simulink model "modelo_BDA"  (R2021b)
settings: Solver=ode3  StartTime=0.0  StopTime=10.0  FixedStep=1e-6  RelTol=1e-3
(part 2 of 4)

== matlab function modelo_BDA/h ==
  data: dq input; h output double; q input
function h = h(dq,q)
%#codegen
dq1 = dq(1);
dq2 = dq(2);
dq3 = dq(3);
dq4 = dq(4);
dq5 = dq(5);
dq6 = dq(6);

q1 = q(1);
q2 = q(2);
q3 = q(3);
q4 = q(4);
q5 = q(5);
q6 = q(6);
%    This function was generated by the Symbolic Math Toolbox version 9.0.
%    01-Dec-2021 19:55:05

t2 = cos(q1);
t3 = cos(q2);
t4 = cos(q4);
t5 = cos(q5);
t6 = cos(q6);
t7 = sin(q1);
t8 = sin(q2);
t9 = sin(q4);
t10 = sin(q5);
t11 = sin(q6);
t12 = dq1+dq2;
t13 = dq5.*6.0;
t20 = dq6.*7.26735103;
t21 = dq1.*2.038587093e+1;
t22 = dq2.*2.038587093e+1;
t23 = dq4.*2.889644336e+1;
t28 = dq5.*1.087689656e+1;
t29 = dq3.*5.110348748545983e-1;
t33 = dq3.*8.595599785252598e-1;
t34 = 9.007199254740992e+15;
t48 = dq6.*1.336375981993753e+2;
t50 = dq6.*7.263507131821755e+1;
t52 = dq4.*6.678442840618982e+2;
t53 = dq5.*6.185536839278779e+1;
t54 = dq5.*1.356524863046341e+2;
t56 = dq4.*1.688943762888624e+2;
t59 = dq3.*1.476709031622059e+1;
t61 = dq3.*1.705746846438843;
t62 = dq5.*7.051076542399408e-1;
t63 = dq3.*2.869063922714997;
t65 = dq4.*1.870703729528352e-1;
t66 = dq6.*1.40259874879e-5;
t84 = dq6.*1.246862890394724e+3;
t87 = dq4.*6.597219446016286e+2;
t88 = dq5.*7.291450524218959e+2;
t90 = dq3.*3.41291720127931e+2;
t94 = dq3.*8.631091645042425e+1;
t99 = dq4.*2.625724653752266e+4;
t100 = dq5.*2.524704765397172;
t101 = dq3.*1.573543358425071e+1;
t103 = dq5.*1.758766552463174e+1;
t104 = dq4.*4.967071763045598;
t105 = dq3.*2.942260910305135e+1;
t109 = dq3.*4.515804268730207e+1;
t110 = dq3.*9.559948463095517e-2;
t111 = dq3.*2.64669783204376e+1;
t112 = dq3.*1.74926470944712e+1;
t116 = dq6.*4.126305645247942e-4;
t117 = dq6.*3.146556876441599e-4;
t118 = dq4.*1.692526621106363;
t124 = dq3.*1.483306048043653e-5;
t125 = dq3.*8.818711196088817e-6;
t126 = dq5.*5.878411097842592e+2;
t127 = dq5.*2.257319383180457e+3;
t129 = dq4.*2.326738990698287e+4;
t130 = dq6.*1.744166601788531e+3;
t131 = dq6.*3.383303336574349e+3;
t132 = dq3.*3.371409213983255e+2;
t135 = dq3.*4.384438618576911e+2;
t138 = dq3.*7.374619913957088e+2;
t147 = dq3.*2.538346896821816;
t148 = dq3.*1.341836869832923e+4;
t150 = dq3.*8.649401300051666e-1;
t162 = dq3.*5.644976860104108e-5;
t163 = dq3.*4.471679626929696e-4;
t164 = dq3.*2.65855123043135e-4;
t165 = dq3.*9.494843556473991e-5;
t166 = dq3.*3.907181940919286e-4;
t171 = dq3.*1.189044768930814e+4;
t176 = dq3.*4.580783722140037e+2;
t177 = dq3.*5.353365437196861e+2;
t14 = t12.^2;
t15 = t2.*t3.*9.81e+3;
t16 = t2.*t8.*9.81e+3;
t17 = t3.*t7.*9.81e+3;
t18 = t7.*t8.*9.81e+3;
t24 = t3.*3.235524933e+1;
t25 = t8.*3.235524933e+1;
t26 = t3.*1.0513390433e+2;
t27 = t8.*1.0513390433e+2;
t30 = t5.*5.110348748545983e-1;
t32 = t10.*5.110348748545983e-1;
t35 = t5.*t9.*8.595599785252598e-1;
t36 = t9.*t10.*8.595599785252598e-1;
t38 = (q3.*t34)./9.007199254740992e+15;
t41 = q3.*t34.*1.110223024625157e-16i;
t67 = -t62;
t68 = t21+t22;
t69 = t7.*t8.*4.486343276457132e+6;
t70 = t2.*t8.*3.161091753815448e+6;
t71 = t3.*t7.*3.161091753815448e+6;
t73 = t2.*t3.*4.486343276457132e+6;
t113 = -t103;
t115 = -t105;
t128 = -t126;
t168 = -t163;
t19 = -t18;
t31 = -t27;
t37 = -t36;
t39 = cos(t38);
t40 = sin(t38);
t42 = exp(t41);
t44 = -t41;
t72 = t25+t26;
t74 = -t69;
t75 = -t70;
t76 = -t71;
t80 = t32+t35;
t43 = t39.^2;
t45 = 1.0./t42;
t46 = t4.*t39;
t47 = t9.*t39;
t51 = t42-1.0;
t77 = t24+t31;
t78 = dq1.*dq2.*t72;
t81 = t30+t37;
t83 = t39.*1.318958611e+1;
t120 = t5.*t12.*t33.*t39;
t122 = t10.*t12.*t33.*t39;
t123 = dq3.*t5.*t12.*t39.*(-8.595599785252598e-1);
t137 = t42.*3.694216783411725e-1;
t145 = t42.*1.305783216588275e-1;
t161 = t12.*t39.*1.72565741205e-5;
t172 = t4.*t34.*t40.*5.673626844500105e-17;
t173 = t9.*t34.*t40.*5.673626844500105e-17;
t174 = t5.*t34.*t40.*9.543032792050485e-17;
t175 = t10.*t34.*t40.*9.543032792050485e-17;
t178 = t4.*t34.*t40.*3.404176106700063e-16;
t181 = t12.*t34.*t40.*5.673626844500105e-17;
t182 = t12.*t34.*t40.*9.543032792050485e-17;
t184 = t42.*3.269483204543573;
t189 = t42.*1.334999662191606e+1;
t192 = t12.*t39.*2.666747250761074e+2;
t193 = dq3.*t10.*t12.*t39.*6.243420034246779e+1;
t196 = dq3.*t12.*t39.*1.451748464558917e+2;
t198 = dq3.*t10.*t12.*t39.*1.148695310384223e+2;
t200 = t12.*t39.*t109;
t202 = dq3.*t10.*t12.*t39.*5.316839912737671e+1;
t212 = dq3.*t12.*t39.*(-4.515804268730207e+1);
t216 = dq3.*t5.*t12.*t39.*1.166014482149094e+2;
t222 = dq3.*t12.*t39.*1.607982057580514e-1;
t227 = t12.*t39.*1.104616756676389e-4;
t228 = dq3.*t5.*t12.*t39.*6.060823201364798e-1;
t229 = dq3.*t10.*t12.*t39.*6.060823201364798e-1;
t230 = t12.*t39.*5.202289239433555e-4;
t231 = t12.*t39.*t125;
t232 = t12.*t39.*t124;
t241 = t4.*t34.*t40.*2.556183965391409e-15;
t242 = t34.*t40.*4.869208971920574e-15;
t243 = t9.*t34.*t40.*9.827649182848514e-15;
t244 = t9.*t34.*t40.*4.958440210927941e-15;
t246 = t4.*t34.*t40.*7.425392937311983e-15;
t248 = t12.*t39.*4.478274624984646e+2;
t249 = t12.*t39.*4.642566765942165e+2;
t250 = t12.*t34.*t40.*2.757597065581095e-15;
t251 = t12.*t34.*t40.*3.18530082611956e-16;
t252 = t12.*t34.*t40.*1.893759423098155e-16;
t256 = dq3.*t12.*t39.*5.670705805344185e+2;
t263 = dq3.*t5.*t12.*t39.*6.267439056015643e+2;
t264 = dq3.*t10.*t12.*t39.*3.610943527871318e+3;
t265 = dq3.*t10.*t12.*t39.*6.267439056015643e+2;
t273 = dq3.*t12.*t39.*4.269496097976898;
t278 = dq3.*t5.*t12.*t39.*2.170135173927414;
t287 = dq3.*t10.*t12.*t39.*1.511765340066191e+1;
t288 = t12.*t39.*t166;
t289 = dq3.*t10.*t12.*t39.*3.54680719181798e-4;
t290 = dq3.*t10.*t12.*t39.*2.704654361142649e-4;
t292 = dq3.*t5.*t12.*t39.*1.940301400531246e+3;
t293 = dq3.*t10.*t12.*t39.*5.052846917024227e+2;
t294 = dq3.*t12.*t39.*3.522681996322863e+3;
t296 = t12.*t34.*t40.*6.373259902786174e-14;
t297 = t12.*t34.*t40.*1.611764571317528e-14;
t298 = t12.*t34.*t40.*1.74698406676951e-15;
t299 = t12.*t34.*t40.*1.942073956592427e-15;
t301 = t12.*t34.*t40.*1.78521870351002e-17;
t303 = t12.*t39.*t176;
t304 = t12.*t34.*t40.*3.266565807075334e-15;
t305 = t12.*t39.*t177;
t306 = t12.*t34.*t40.*2.938424872360468e-15;
t307 = t12.*t34.*t40.*9.963509157680404e-16;
t309 = dq3.*t12.*t39.*(-5.353365437196861e+2);
t312 = t12.*t34.*t40.*9.790736217417458e-22;
t315 = t12.*t34.*t40.*1.646800527103812e-21;
t318 = t34.*t40.*t72.*5.673626844500105e-17;
t344 = t12.*t34.*t40.*4.867704704399801e-14;
t345 = t12.*t34.*t40.*8.18747282633435e-14;
t346 = t12.*t34.*t40.*6.295748150968656e-14;
t348 = t12.*t34.*t40.*2.505737647365328e-12;
t350 = t12.*t34.*t40.*4.740092871521216e-16;
t351 = t12.*t34.*t40.*6.267183283563802e-21;
t352 = t12.*t34.*t40.*1.054139393161123e-20;
t353 = t12.*t34.*t40.*1.615183704663643e-16;
t355 = t12.*t34.*t40.*2.951584788170425e-20;
t357 = t12.*t34.*t40.*4.005724181331548e-20;
t358 = t12.*t34.*t40.*4.964561680564579e-20;
t375 = t12.*t34.*t40.*2.220414648677621e-12;
t402 = t12.*t34.*t40.*8.913349685100906e-16;
t406 = t12.*t34.*t40.*2.760619280862119e-14;
t49 = t47.*6.0;
t55 = t12.*t46;
t57 = t12.*t47;
t58 = t51.^2;
t79 = dq1.*dq2.*t77;
t85 = t46.*2.286892447e+1;
t86 = t47.*2.286892447e+1;
t89 = t12.*t83;
t91 = t46.*6.520967601e+1;
t92 = t15+t19+t78;
t146 = t45.*3.694216783411725e-1;
t152 = t45.*1.305783216588275e-1;
t155 = t14.*t43.*3.422984996757468e+1;
t157 = t14.*t43.*3.079131064925427e+1;
t167 = -t161;
t169 = t78.*4.573234736449676e+2;
t179 = -t173;
t180 = -t174;
t183 = -t181;
t185 = t45.*3.269483204543573;
t195 = t45.*1.334999662191606e+1;
t199 = -t192;
t201 = -t193;
t204 = -t196;
t223 = -t216;
t245 = -t243;
t247 = t12.*t242;
t253 = -t252;
t254 = t29+t182;
t267 = -t263;
t268 = -t264;
t269 = -t265;
t277 = -t273;
t291 = -t290;
t300 = -t298;
t302 = t47+t172;
t316 = -t312;
t319 = t34.*t40.*t77.*9.543032792050485e-17;
t320 = dq1.*t318;
t325 = dq1.*t34.*t40.*t77.*(-9.543032792050485e-17);
t347 = -t344;
t356 = -t351;
t361 = -t357;
t363 = t61+t251;
t403 = -t402;
t417 = t23+t59+t250;
t491 = t112+t304;
t492 = t109+t307;
t502 = t125+t315;
t604 = t56+t94+t297;
t610 = t65+t110+t301;
t624 = t176+t406;
t630 = t115+t161+t299;
t701 = t135+t230+t345;
t704 = t168+t192+t355;
t746 = t164+t249+t358;
t60 = t12.*t49;
t64 = -t57;
t82 = -t79;
t93 = -t91;
t95 = t55.*2.889644336e+1;
t96 = t57.*2.889644336e+1;
t97 = t55.*2.286892447e+1;
t98 = t57.*2.286892447e+1;
t102 = t55.*6.520967601e+1;
t107 = t57.*1.087689656e+1;
t114 = t29.*t57;
t119 = t29.*t55;
t121 = dq3.*t57.*(-5.110348748545983e-1);
t133 = t55.*6.678442840618982e+2;
t134 = t57.*6.678442840618982e+2;
t136 = dq3.*t55.*2.302405830805438e+1;
t139 = t57.*6.185536839278779e+1;
t140 = t55.*1.688943762888624e+2;
t141 = dq3.*t55.*2.228321894484292e+1;
t142 = t57.*1.356524863046341e+2;
t143 = t57.*1.688943762888624e+2;
t149 = dq3.*t57.*4.466165897254792e+1;
t153 = t57.*7.051076542399408e-1;
t154 = t55.*1.870703729528352e-1;
t156 = t57.*1.870703729528352e-1;
t170 = t79.*3.22231575312482e+2;
t186 = t55.*6.597219446016286e+2;
t187 = t57.*6.597219446016286e+2;
t188 = t57.*7.291450524218959e+2;
t191 = dq3.*t55.*4.097608396301209e+2;
t194 = dq3.*t55.*2.227143274869608e+2;
t197 = dq3.*t57.*4.857802448423996e+2;
t203 = t57.*t94;
t206 = t57.*2.625724653752266e+4;
t207 = dq3.*t55.*3.161025044569338e+1;
t208 = dq3.*t55.*6.932315136240378e+1;
t209 = t57.*2.524704765397172;
t210 = dq3.*t55.*1.006605116943962e+3;
t211 = dq3.*t57.*1.006605116943962e+3;
t213 = t57.*1.758766552463174e+1;
t214 = t55.*4.967071763045598;
t215 = t57.*4.967071763045598;
t224 = t55.*1.692526621106363;
t225 = t57.*1.692526621106363;
t226 = t55.*t110;
t233 = t57.*5.878411097842592e+2;
t234 = t57.*2.257319383180457e+3;
t236 = t55.*4.098238731829628e+3;
t237 = t57.*4.098238731829628e+3;
t238 = t55.*2.326738990698287e+4;
t255 = dq4+t254;
t257 = t33+t183;
t258 = dq3.*t55.*1.359241913128349e+3;
t259 = dq3.*t57.*6.058465082115794e+3;
t260 = dq3.*t57.*2.762563368780008e+3;
t270 = dq3.*t55.*4.225774888975571e+3;
t276 = dq3.*t57.*2.87948544352712e+4;
t279 = dq3.*t57.*6.845466071397372;
t280 = dq3.*t55.*8.987910450364716;
t281 = dq3.*t55.*1.290212183829552;
t282 = t55.*t150;
t283 = t57.*t150;
t295 = dq3.*t55.*2.726693342625011e+4;
t308 = t46+t179;
t310 = t6.*t302;
t311 = t11.*t302;
t321 = -t319;
t322 = dq1.*t319;
t323 = t4.*t254.*1.318958611e+1;
t324 = t9.*t254.*1.318958611e+1;
t328 = t33.*t254;
t330 = t45.*t58.*5.499266393288274;
t332 = dq3.*t254.*(-8.595599785252598e-1);
t341 = t45.*t58.*7.936984065608979;
t349 = t34.*t40.*t92.*9.543032792050485e-17;
t360 = t5.*t302.*4.234075154e+1;
t362 = t10.*t302.*4.234075154e+1;
t364 = t63+t253;
t367 = dq3.*t254.*1.133724035346867e+1;
t408 = t45.*t58.*t72.*2.196325630278387e-1;
t409 = t45.*t58.*t77.*2.196325630278387e-1;
t413 = dq1.*t45.*t58.*t77.*(-2.196325630278387e-1);
t414 = t34.*t40.*t92.*3.18530082611956e-16;
t418 = dq3.*t254.*3.276059237327137e+2;
t429 = t105.*t254;
t431 = t111.*t254;
t435 = dq3.*t254.*(-2.64669783204376e+1);
t458 = t45.*t58.*t92.*2.196325630278387e-1;
t482 = t34.*t40.*t92.*3.266565807075334e-15;
t483 = t34.*t40.*t92.*2.938424872360468e-15;
t490 = t111+t300;
t493 = dq3.*t254.*1.914796138336013e+3;
t495 = t138.*t254;
t497 = dq3.*t254.*2.120861781179316;
t503 = t165.*t254;
t504 = t163.*t254;
t505 = t124+t316;
t506 = dq3.*t254.*(-9.494843556473991e-5);
t508 = dq3.*t254.*(-4.471679626929696e-4);
t517 = t45.*t58.*t92.*7.330958613472507e-1;
t531 = t137+t146+2.61156643317655e-1;
t536 = t145+t152+7.38843356682345e-1;
t551 = t45.*t58.*t92.*6.762774476882097;
t577 = t45.*t58.*t92.*3.790105603165286e-6;
t605 = t12.*t39.*t492;
t613 = t166+t361;
t623 = t177+t403;
t628 = t101+t167+t306;
t668 = t254.*t491;
t670 = t254.*t502;
t702 = t138+t227+t347;
t703 = t162+t199+t352;
t745 = t165+t248+t356;
t756 = t12.*t39.*t701;
t765 = t247+t320+t325;
t769 = t254.*t630;
t800 = t254.*t704;
t806 = t254.*t746;
t106 = t16+t17+t82;
t108 = -t96;
t144 = -t134;
t151 = -t143;
t158 = -t153;
t159 = -t154;
t160 = -t156;
t190 = -t187;
t205 = -t197;
t217 = -t210;
t218 = -t211;
t219 = -t213;
t220 = -t214;
t221 = -t215;
t235 = -t233;
t239 = -t236;
t240 = -t237;
t261 = t5.*t255;
t262 = t10.*t255;
t266 = -t260;
t271 = t4.*t257;
t272 = t9.*t257;
t286 = -t279;
t313 = t5.*t308;
t314 = t10.*t308;
t317 = -t311;
t327 = -t324;
t331 = t29.*t257;
t372 = dq3.*t257.*6.740338487107798;
t410 = dq1.*t408;
t411 = -t409;
t412 = dq1.*t409;
t415 = -t414;
t424 = dq3.*t257.*1.947718093199386e+2;
t436 = t101.*t257;
t438 = t112.*t257;
t448 = dq3.*t257.*(-1.74926470944712e+1);
t460 = -t458;
t485 = -t482;
t494 = dq3.*t257.*1.138405264755886e+3;
t498 = t135.*t257;
t499 = dq3.*t257.*(-4.384438618576911e+2);
t500 = dq3.*t257.*1.260917634611605;
t507 = t162.*t257;
t514 = t164.*t257;
t557 = -t551;
t583 = -t577;
t617 = t72.*t536;
t618 = t77.*t531;
t625 = t92.*t531;
t629 = t12.*t39.*t613;
t669 = t257.*t490;
t671 = t257.*t505;
t744 = t255.*t604;
t747 = t255.*t610;
t757 = t12.*t39.*t702;
t758 = -t756;
t759 = t254.*t623;
t761 = t257.*t624;
t762 = t242+t318+t321;
t766 = t4.*t765;
t767 = t9.*t765;
t770 = t184+t185+t341+1.849951749091285e+1;
t771 = t257.*t628;
t775 = t189+t195+t330+9.437562846167879;
t784 = t29.*t765;
t785 = t33.*t765;
t786 = dq3.*t765.*2.483822623397798e+1;
t787 = t63.*t765;
t788 = t61.*t765;
t789 = dq3.*t765.*(-1.705746846438843);
t793 = dq3.*t765.*1.451748464558917e+2;
t794 = t109.*t765;
t796 = dq3.*t765.*1.607982057580514e-1;
t797 = t124.*t765;
t799 = t125.*t765;
t801 = t257.*t703;
t807 = t12.*t39.*t765.*3.422984996757468e+1;
t808 = t12.*t39.*t765.*3.079131064925427e+1;
t809 = t257.*t745;
t837 = t363.*t765;
t838 = t364.*t765;
t893 = t492.*t765;
t274 = -t261;
t275 = t271.*6.0;
t284 = -t271;
t326 = t262.*7.26735103;
t329 = t262.*1.087689656e+1;
t333 = t271.*2.889644336e+1;
t334 = t272.*2.889644336e+1;
t335 = t271.*2.286892447e+1;
t336 = t272.*2.286892447e+1;
t337 = t261.*1.087689656e+1;
t338 = t272.*6.520967601e+1;
t339 = t271.*1.087689656e+1;
t354 = t34.*t40.*t106.*5.673626844500105e-17;
t365 = t262.*7.263507131821755e+1;
t366 = t262.*1.336375981993753e+2;
t368 = t272.*6.678442840618982e+2;
t369 = t261.*1.356524863046341e+2;
t370 = t262.*1.356524863046341e+2;
t371 = t261.*6.185536839278779e+1;
t373 = t262.*6.185536839278779e+1;
t374 = t271.*6.678442840618982e+2;
t377 = t271.*6.185536839278779e+1;
t379 = t271.*1.356524863046341e+2;
t380 = -t372;
t381 = t271.*1.688943762888624e+2;
t382 = t272.*1.688943762888624e+2;
t383 = t261.*7.051076542399408e-1;
t384 = t262.*7.051076542399408e-1;
t389 = t271.*7.051076542399408e-1;
t390 = t262.*1.40259874879e-5;
t391 = t55+t272;
t392 = t271.*1.870703729528352e-1;
t393 = t272.*1.870703729528352e-1;
t396 = t64+t271;
t416 = t34.*t40.*t106.*1.893759423098155e-16;
t419 = t261.*7.291450524218959e+2;
t420 = t262.*7.291450524218959e+2;
t421 = t262.*1.246862890394724e+3;
t422 = t261.*2.65978307941329e+3;
t423 = t262.*2.65978307941329e+3;
t426 = t271.*6.597219446016286e+2;
t427 = t271.*7.291450524218959e+2;
t428 = t272.*6.597219446016286e+2;
t430 = -t424;
t433 = t261.*2.524704765397172;
h = ft_1({dq1,dq2,dq3,dq4,dq5,dq6,t10,t100,t101,t102,t103,t104,t105,t106,t107,t108,t11,t111,t112,t113,t116,t117,t118,t119,t12,t120,t121,t122,t123,t126,t127,t128,t129,t13,t130,t131,t132,t133,t134,t136,t139,t140,t141,t142,t143,t144,t147,t148,t149,t150,t151,t153,t154,t155,t156,t157,t158,t159,t160,t169,t170,t171,t174,t175,t178,t180,t186,t188,t190,t191,t194,t196,t197,t198,t2,t20,t201,t202,t203,t204,t205,t206,t207,t208,t209,t210,t211,t212,t215,t216,t217,t218,t219,t220,t221,t222,t223,t224,t225,t226,t228,t229,t23,t231,t232,t234,t235,t238,t239,t240,t241,t244,t245,t246,t254,t255,t256,t257,t258,t259,t261,t262,t264,t266,t267,t268,t269,t270,t271,t272,t274,t275,t276,t277,t278,t28,t280,t281,t282,t283,t284,t286,t287,t288,t289,t29,t291,t292,t293,t294,t295,t296,t3,t302,t303,t305,t308,t309,t310,t311,t313,t314,t317,t323,t326,t327,t328,t329,t33,t331,t332,t333,t334,t335,t336,t337,t338,t339,t34,t346,t348,t349,t350,t353,t354,t360,t362,t363,t364,t365,t366,t367,t368,t369,t370,t371,t373,t374,t375,t377,t379,t380,t381,t382,t383,t384,t389,t39,t390,t391,t392,t393,t4,t40,t408,t410,t411,t413,t415,t416,t417,t418,t419,t420,t421,t422,t423,t426,t427,t428,t429,t430,t433,t435,t436,t448,t45,t460,t48,t482,t483,t485,t49,t490,t491,t493,t494,t495,t497,t499,t5,t50,t500,t502,t504,t505,t506,t507,t508,t514,t517,t52,t53,t536,t54,t55,t557,t56,t57,t577,t58,t583,t6,t60,t604,t605,t61,t610,t617,t618,t62,t625,t628,t629,t63,t630,t65,t66,t668,t669,t67,t670,t671,t68,t7,t72,t73,t74,t744,t747,t75,t756,t757,t758,t759,t76,t761,t762,t765,t766,t767,t769,t77,t770,t771,t775,t78,t784,t785,t786,t787,t789,t79,t793,t794,t796,t797,t799,t8,t80,t800,t801,t806,t807,t808,t809,t81,t83,t837,t838,t84,t85,t86,t87,t88,t89,t893,t9,t90,t91,t92,t93,t95,t96,t97,t98,t99});
end
function h = ft_1(ct)
dq1 = ct{1};
dq2 = ct{2};
dq3 = ct{3};
dq4 = ct{4};
dq5 = ct{5};
dq6 = ct{6};
t10 = ct{7};
t100 = ct{8};
t101 = ct{9};
t102 = ct{10};
t103 = ct{11};
t104 = ct{12};
t105 = ct{13};
t106 = ct{14};
t107 = ct{15};
t108 = ct{16};
t11 = ct{17};
t111 = ct{18};
t112 = ct{19};
t113 = ct{20};
t116 = ct{21};
t117 = ct{22};
t118 = ct{23};
t119 = ct{24};
t12 = ct{25};
t120 = ct{26};
t121 = ct{27};
t122 = ct{28};
t123 = ct{29};
t126 = ct{30};
t127 = ct{31};
t128 = ct{32};
t129 = ct{33};
t13 = ct{34};
t130 = ct{35};
t131 = ct{36};
t132 = ct{37};
t133 = ct{38};
t134 = ct{39};
t136 = ct{40};
t139 = ct{41};
t140 = ct{42};
t141 = ct{43};
t142 = ct{44};
t143 = ct{45};
t144 = ct{46};
t147 = ct{47};
t148 = ct{48};
t149 = ct{49};
t150 = ct{50};
t151 = ct{51};
t153 = ct{52};
t154 = ct{53};
t155 = ct{54};
t156 = ct{55};
t157 = ct{56};
t158 = ct{57};
t159 = ct{58};
t160 = ct{59};
t169 = ct{60};
t170 = ct{61};
t171 = ct{62};
t174 = ct{63};
t175 = ct{64};
t178 = ct{65};
t180 = ct{66};
t186 = ct{67};
t188 = ct{68};
t190 = ct{69};
t191 = ct{70};
t194 = ct{71};
t196 = ct{72};
t197 = ct{73};
t198 = ct{74};
t2 = ct{75};
t20 = ct{76};
t201 = ct{77};
t202 = ct{78};
t203 = ct{79};
t204 = ct{80};
t205 = ct{81};
t206 = ct{82};
t207 = ct{83};
t208 = ct{84};
t209 = ct{85};
t210 = ct{86};
t211 = ct{87};
t212 = ct{88};
t215 = ct{89};
t216 = ct{90};
t217 = ct{91};
t218 = ct{92};
t219 = ct{93};
t220 = ct{94};
t221 = ct{95};
t222 = ct{96};
t223 = ct{97};
t224 = ct{98};
t225 = ct{99};
t226 = ct{100};
t228 = ct{101};
t229 = ct{102};
t23 = ct{103};
t231 = ct{104};
t232 = ct{105};
t234 = ct{106};
t235 = ct{107};
t238 = ct{108};
t239 = ct{109};
t240 = ct{110};
t241 = ct{111};
t244 = ct{112};
t245 = ct{113};
t246 = ct{114};
t254 = ct{115};
t255 = ct{116};
t256 = ct{117};
t257 = ct{118};
t258 = ct{119};
t259 = ct{120};
t261 = ct{121};
t262 = ct{122};
t264 = ct{123};
t266 = ct{124};
t267 = ct{125};
t268 = ct{126};
t269 = ct{127};
t270 = ct{128};
t271 = ct{129};
t272 = ct{130};
t274 = ct{131};
t275 = ct{132};
t276 = ct{133};
t277 = ct{134};
t278 = ct{135};
t28 = ct{136};
t280 = ct{137};
t281 = ct{138};
t282 = ct{139};
t283 = ct{140};
t284 = ct{141};
t286 = ct{142};
t287 = ct{143};
t288 = ct{144};
t289 = ct{145};
t29 = ct{146};
t291 = ct{147};
t292 = ct{148};
t293 = ct{149};
t294 = ct{150};
t295 = ct{151};
t296 = ct{152};
t3 = ct{153};
t302 = ct{154};
t303 = ct{155};
t305 = ct{156};
t308 = ct{157};
t309 = ct{158};
t310 = ct{159};
t311 = ct{160};
t313 = ct{161};
t314 = ct{162};
t317 = ct{163};
t323 = ct{164};
t326 = ct{165};
t327 = ct{166};
t328 = ct{167};
t329 = ct{168};
t33 = ct{169};
t331 = ct{170};
t332 = ct{171};
t333 = ct{172};
t334 = ct{173};
t335 = ct{174};
t336 = ct{175};
t337 = ct{176};
t338 = ct{177};
t339 = ct{178};
t34 = ct{179};
t346 = ct{180};
t348 = ct{181};
t349 = ct{182};
t350 = ct{183};
t353 = ct{184};
t354 = ct{185};
t360 = ct{186};
t362 = ct{187};
t363 = ct{188};
t364 = ct{189};
t365 = ct{190};
t366 = ct{191};
t367 = ct{192};
t368 = ct{193};
t369 = ct{194};
t370 = ct{195};
t371 = ct{196};
t373 = ct{197};
t374 = ct{198};
t375 = ct{199};
t377 = ct{200};
t379 = ct{201};
t380 = ct{202};
t381 = ct{203};
t382 = ct{204};
t383 = ct{205};
t384 = ct{206};
t389 = ct{207};
t39 = ct{208};
t390 = ct{209};
t391 = ct{210};
t392 = ct{211};
t393 = ct{212};
t4 = ct{213};
t40 = ct{214};
t408 = ct{215};
t410 = ct{216};
t411 = ct{217};
t413 = ct{218};
t415 = ct{219};
t416 = ct{220};
t417 = ct{221};
t418 = ct{222};
t419 = ct{223};
t420 = ct{224};
t421 = ct{225};
t422 = ct{226};
t423 = ct{227};
t426 = ct{228};
t427 = ct{229};
t428 = ct{230};
t429 = ct{231};
t430 = ct{232};
t433 = ct{233};
t435 = ct{234};
t436 = ct{235};
t448 = ct{236};
t45 = ct{237};
t460 = ct{238};
t48 = ct{239};
t482 = ct{240};
t483 = ct{241};
t485 = ct{242};
t49 = ct{243};
t490 = ct{244};
t491 = ct{245};
t493 = ct{246};
t494 = ct{247};
t495 = ct{248};
t497 = ct{249};
t499 = ct{250};
t5 = ct{251};
t50 = ct{252};
t500 = ct{253};
t502 = ct{254};
t504 = ct{255};
t505 = ct{256};
t506 = ct{257};
t507 = ct{258};
t508 = ct{259};
t514 = ct{260};
t517 = ct{261};
t52 = ct{262};
t53 = ct{263};
t536 = ct{264};
t54 = ct{265};
t55 = ct{266};
t557 = ct{267};
t56 = ct{268};
t57 = ct{269};
t577 = ct{270};
t58 = ct{271};
t583 = ct{272};
t6 = ct{273};
t60 = ct{274};
t604 = ct{275};
t605 = ct{276};
t61 = ct{277};
t610 = ct{278};
t617 = ct{279};
t618 = ct{280};
t62 = ct{281};
t625 = ct{282};
t628 = ct{283};
t629 = ct{284};
t63 = ct{285};
t630 = ct{286};
t65 = ct{287};
t66 = ct{288};
t668 = ct{289};
t669 = ct{290};
t67 = ct{291};
t670 = ct{292};
t671 = ct{293};
t68 = ct{294};
t7 = ct{295};
t72 = ct{296};
t73 = ct{297};
t74 = ct{298};
t744 = ct{299};
t747 = ct{300};
t75 = ct{301};
t756 = ct{302};
t757 = ct{303};
t758 = ct{304};
t759 = ct{305};
t76 = ct{306};
t761 = ct{307};
t762 = ct{308};
t765 = ct{309};
t766 = ct{310};
t767 = ct{311};
t769 = ct{312};
t77 = ct{313};
t770 = ct{314};
t771 = ct{315};
t775 = ct{316};
t78 = ct{317};
t784 = ct{318};
t785 = ct{319};
t786 = ct{320};
t787 = ct{321};
t789 = ct{322};
t79 = ct{323};
t793 = ct{324};
t794 = ct{325};
t796 = ct{326};
t797 = ct{327};
t799 = ct{328};
t8 = ct{329};
t80 = ct{330};
t800 = ct{331};
t801 = ct{332};
t806 = ct{333};
t807 = ct{334};
t808 = ct{335};
t809 = ct{336};
t81 = ct{337};
t83 = ct{338};
t837 = ct{339};
t838 = ct{340};
t84 = ct{341};
t85 = ct{342};
t86 = ct{343};
t87 = ct{344};
t88 = ct{345};
t89 = ct{346};
t893 = ct{347};
t9 = ct{348};
t90 = ct{349};
t91 = ct{350};
t92 = ct{351};
t93 = ct{352};
t95 = ct{353};
t96 = ct{354};
t97 = ct{355};
t98 = ct{356};
t99 = ct{357};
t434 = t262.*2.524704765397172;
t439 = t261.*1.758766552463174e+1;
t440 = t262.*1.758766552463174e+1;
t441 = t271.*2.625724653752266e+4;
t442 = t271.*2.524704765397172;
t443 = t262.*4.126305645247942e-4;
t444 = t271.*1.758766552463174e+1;
t445 = t271.*4.967071763045598;
t446 = t272.*4.967071763045598;
t447 = t262.*3.146556876441599e-4;
t454 = t271.*1.692526621106363;
t455 = t272.*1.692526621106363;
t461 = t261.*5.878411097842592e+2;
t462 = t45.*t58.*t106.*2.196325630278387e-1;
t465 = t271.*5.878411097842592e+2;
t467 = t262.*2.257319383180457e+3;
t470 = t271.*2.257319383180457e+3;
t478 = t271.*4.098238731829628e+3;
t479 = t272.*4.098238731829628e+3;
t480 = t272.*2.326738990698287e+4;
t484 = t34.*t40.*t106.*1.74698406676951e-15;
t486 = t262.*1.744166601788531e+3;
t487 = t262.*3.383303336574349e+3;
t488 = t34.*t40.*t106.*1.942073956592427e-15;
t496 = -t494;
t501 = -t500;
t515 = t45.*t58.*t106.*6.34659991754557;
t529 = t45.*t58.*t106.*7.330958613472507e-1;
t555 = t45.*t58.*t106.*3.709470474531108e+1;
t560 = t45.*t58.*t106.*7.517989680436807;
t566 = t45.*t58.*t106.*4.108674547820486e-2;
t585 = t45.*t58.*t106.*3.790105603165286e-6;
t598 = t175+t313;
t599 = t180+t314;
t600 = -t6.*(t174-t314);
t602 = -t11.*(t174-t314);
t619 = dq1.*t617;
t620 = dq1.*t618;
t621 = -t618;
t626 = t106.*t536;
t627 = -t625;
t631 = t331+t332;
t634 = -t4.*(t328-t331);
t635 = -t9.*(t328-t331);
t639 = t625.*2.889644336e+1;
t641 = t625.*3.33782865;
t652 = t9.*(t328-t331).*(-4.360410618e+1);
t653 = t9.*(t328-t331).*(-2.286892447e+1);
t654 = t4.*(t328-t331).*(-6.520967601e+1);
t655 = t4.*(t328-t331).*6.520967601e+1;
t656 = t625.*1.688943762888624e+2;
t657 = t625.*3.422984996757468e+1;
t660 = t625.*1.870703729528352e-1;
t665 = t625.*1.72565741205e-5;
t672 = t9.*(t328-t331).*(-4.358104279093053e+2);
t673 = t4.*(t328-t331).*(-1.328674864713371e+3);
t674 = t9.*(t328-t331).*(-1.328674864713371e+3);
t675 = t9.*(t328-t331).*(-8.018255891962515e+2);
t676 = t9.*(t328-t331).*1.328674864713371e+3;
t677 = t4.*(t328-t331).*(-1.688943762888624e+2);
t678 = t9.*(t328-t331).*(-1.356524863046341e+2);
t679 = t9.*(t328-t331).*(-6.185536839278779e+1);
t680 = t4.*(t328-t331).*1.688943762888624e+2;
t681 = t4.*(t328-t331).*(-7.092789006718835e+2);
t685 = t9.*(t328-t331).*(-1.870703729528352e-1);
t705 = t9.*(t328-t331).*(-4.522154679359383e+3);
t706 = t9.*(t328-t331).*(-2.65978307941329e+3);
t707 = t4.*(t328-t331).*(-4.033568532372886e+3);
t708 = t4.*(t328-t331).*(-8.84585468187615e+3);
t709 = t4.*(t328-t331).*8.84585468187615e+3;
t710 = t9.*(t328-t331).*(-2.524704765397172);
t712 = t4.*(t328-t331).*(-9.245169992678717);
t713 = t4.*(t328-t331).*(-4.153012702745543e+4);
t715 = t9.*(t328-t331).*(-1.758766552463174e+1);
t716 = t4.*(t328-t331).*(-1.692526621106363);
t717 = t9.*(t328-t331).*(-1.692526621106363);
t718 = t4.*(t328-t331).*4.153012702745543e+4;
t721 = t4.*(t328-t331).*1.692526621106363;
t740 = t9.*(t328-t331).*(-3.854027039691565e+4);
t760 = -t759;
t763 = t9.*t762;
t764 = t4.*t762;
t768 = -t767;
t772 = -t771;
t773 = t4.*t770;
t774 = t9.*t770;
t777 = t12.*t770;
t779 = t12.*t775;
t802 = t83+t775;
t810 = -t809;
t841 = -t838;
t894 = -t893;
t934 = t411+t617+t770;
t285 = -t275;
t340 = -t335;
t342 = -t337;
t343 = -t339;
t359 = -t354;
t376 = -t369;
t378 = -t371;
t385 = -t377;
t386 = -t379;
t387 = -t381;
t388 = -t383;
t394 = -t389;
t395 = -t393;
t397 = dq4.*t391;
t398 = t5.*t391;
t399 = t10.*t391;
t400 = dq5+t57+t284;
t401 = -dq4.*(t57+t284);
t425 = -t422;
t432 = -t427;
t437 = -t433;
t449 = -t439;
t450 = -t441;
t451 = -t442;
t452 = -t445;
t453 = -t446;
t456 = -t454;
t463 = dq4.*(t57+t284).*(-4.234075154e+1);
t468 = t5.*(t57+t284).*(-4.234075154e+1);
t469 = t10.*(t57+t284).*(-4.234075154e+1);
t471 = dq4.*(t57+t284).*4.234075154e+1;
t474 = t5.*(t57+t284).*4.234075154e+1;
t475 = t10.*(t57+t284).*4.234075154e+1;
t476 = -t470;
t481 = -t479;
t489 = -t484;
t510 = t95+t334;
t513 = t52.*t391;
t519 = t108+t333;
t522 = dq4.*(t57+t284).*(-4.605359747732407e+2);
t527 = dq4.*(t57+t284).*(-6.678442840618982e+2);
t535 = dq4.*(t57+t284).*(-1.688943762888624e+2);
t539 = t65.*t391;
t541 = t56.*(t57+t284);
t548 = t87.*t391;
t558 = dq4.*(t57+t284).*(-2.619002784534197e+3);
t559 = dq4.*(t57+t284).*(-5.743628218407764e+3);
t561 = dq4.*(t57+t284).*5.743628218407764e+3;
t573 = dq4.*(t57+t284).*(-2.625724653752266e+4);
t574 = t118.*t391;
t579 = dq4.*(t57+t284).*(-4.967071763045598);
t581 = t99.*(t57+t284);
t584 = dq4.*(t57+t284).*(-1.692526621106363);
t587 = t118.*(t57+t284);
t597 = t129.*t391;
t601 = t6.*t598.*6.0;
t603 = t11.*t598.*6.0;
t612 = t133+t368;
t614 = t144+t374;
t615 = t140+t382;
t616 = t160+t392;
t622 = -t620;
t642 = -t639;
t645 = -t641;
t649 = t626.*3.33782865;
t658 = -t656;
t659 = -t657;
t661 = t626.*3.079131064925427e+1;
t664 = -t660;
t666 = -t665;
t667 = t626.*1.72565741205e-5;
t754 = t310+t602;
t755 = t317+t600;
t782 = (t57+t284).*(t134-t374);
t783 = (t57+t284).*(t156-t392);
t803 = t5.*t802;
t804 = t10.*t802;
t811 = t52+t90+t151+t296+t381;
t823 = -t5.*(dq4.*(t57+t284)+dq3.*t57.*5.110348748545983e-1+t4.*(t328-t331));
t824 = -t10.*(dq4.*(t57+t284)+dq3.*t57.*5.110348748545983e-1+t4.*(t328-t331));
t845 = t5.*(dq4.*(t57+t284)+dq3.*t57.*5.110348748545983e-1+t4.*(t328-t331)).*(-1.336375981993753e+2);
t846 = t5.*(dq4.*(t57+t284)+dq3.*t57.*5.110348748545983e-1+t4.*(t328-t331)).*(-7.263507131821755e+1);
t847 = t5.*(dq4.*(t57+t284)+dq3.*t57.*5.110348748545983e-1+t4.*(t328-t331)).*7.263507131821755e+1;
t848 = t5.*(dq4.*(t57+t284)+dq3.*t57.*5.110348748545983e-1+t4.*(t328-t331)).*(-6.185536839278779e+1);
t851 = t10.*(dq4.*(t57+t284)+dq3.*t57.*5.110348748545983e-1+t4.*(t328-t331)).*(-1.356524863046341e+2);
t852 = t5.*(dq4.*(t57+t284)+dq3.*t57.*5.110348748545983e-1+t4.*(t328-t331)).*(-7.051076542399408e-1);
t853 = t10.*(dq4.*(t57+t284)+dq3.*t57.*5.110348748545983e-1+t4.*(t328-t331)).*(-7.051076542399408e-1);
t854 = t10.*(dq4.*(t57+t284)+dq3.*t57.*5.110348748545983e-1+t4.*(t328-t331)).*7.051076542399408e-1;
t855 = t186+t221+t428+t445;
t865 = t5.*(dq4.*(t57+t284)+dq3.*t57.*5.110348748545983e-1+t4.*(t328-t331)).*(-7.291450524218959e+2);
t866 = t10.*(dq4.*(t57+t284)+dq3.*t57.*5.110348748545983e-1+t4.*(t328-t331)).*(-7.291450524218959e+2);
t867 = t86+t246+t774;
t868 = t5.*(dq4.*(t57+t284)+dq3.*t57.*5.110348748545983e-1+t4.*(t328-t331)).*(-4.200920957332826e+3);
t869 = t5.*(dq4.*(t57+t284)+dq3.*t57.*5.110348748545983e-1+t4.*(t328-t331)).*7.291450524218959e+2;
t870 = t5.*(dq4.*(t57+t284)+dq3.*t57.*5.110348748545983e-1+t4.*(t328-t331)).*4.200920957332826e+3;
t872 = t91+t245+t773;
t875 = t10.*(dq4.*(t57+t284)+dq3.*t57.*5.110348748545983e-1+t4.*(t328-t331)).*(-2.524704765397172);
t876 = t5.*(dq4.*(t57+t284)+dq3.*t57.*5.110348748545983e-1+t4.*(t328-t331)).*(-1.758766552463174e+1);
t879 = t10.*(dq4.*(t57+t284)+dq3.*t57.*5.110348748545983e-1+t4.*(t328-t331)).*2.524704765397172;
t880 = t5.*(dq4.*(t57+t284)+dq3.*t57.*5.110348748545983e-1+t4.*(t328-t331)).*(-4.126305645247942e-4);
t881 = t5.*(dq4.*(t57+t284)+dq3.*t57.*5.110348748545983e-1+t4.*(t328-t331)).*(-3.146556876441599e-4);
t882 = t5.*(dq4.*(t57+t284)+dq3.*t57.*5.110348748545983e-1+t4.*(t328-t331)).*3.146556876441599e-4;
t883 = t118+t150+t186+t353+t428;
t884 = t5.*(dq4.*(t57+t284)+dq3.*t57.*5.110348748545983e-1+t4.*(t328-t331)).*(-5.878411097842592e+2);
t885 = t10.*(dq4.*(t57+t284)+dq3.*t57.*5.110348748545983e-1+t4.*(t328-t331)).*(-2.257319383180457e+3);
t886 = t10.*(dq4.*(t57+t284)+dq3.*t57.*5.110348748545983e-1+t4.*(t328-t331)).*2.257319383180457e+3;
t892 = t87+t132+t240+t346+t478;
t896 = t129+t171+t190+t375+t426;
t935 = t4.*t934;
t936 = t9.*t934;
t938 = t413+t619+t777;
t946 = t460+t626+t784;
t954 = t408+t621+t802;
t1062 = t367+t380+t462+t627+t785;
t404 = t6.*t400;
t405 = t11.*t400;
t457 = t397.*4.360410618e+1;
t459 = t398.*7.26735103;
t464 = t398.*1.087689656e+1;
t466 = t399.*1.087689656e+1;
t509 = t398.*7.263507131821755e+1;
t511 = t397.*4.358104279093053e+2;
t512 = t398.*1.336375981993753e+2;
t516 = t397.*8.018255891962515e+2;
t518 = t397.*6.185536839278779e+1;
t520 = t397.*1.356524863046341e+2;
t521 = t397.*(-6.678442840618982e+2);
t523 = t398.*1.356524863046341e+2;
t524 = t399.*1.356524863046341e+2;
t525 = t398.*6.185536839278779e+1;
t526 = t399.*6.185536839278779e+1;
t537 = t399.*7.051076542399408e-1;
t542 = t398.*7.051076542399408e-1;
t543 = t398.*1.40259874879e-5;
t547 = t397.*2.65978307941329e+3;
t549 = t398.*7.291450524218959e+2;
t550 = t399.*7.291450524218959e+2;
t552 = t398.*1.246862890394724e+3;
t553 = t398.*2.65978307941329e+3;
t554 = t399.*2.65978307941329e+3;
t562 = t397.*2.524704765397172;
t563 = t397.*1.758766552463174e+1;
t564 = t398.*2.524704765397172;
t565 = t399.*2.524704765397172;
t571 = t398.*1.758766552463174e+1;
t572 = t399.*1.758766552463174e+1;
t578 = t398.*3.146556876441599e-4;
t582 = t398.*4.126305645247942e-4;
t586 = t28+t107+t343;
t594 = t399.*5.878411097842592e+2;
t596 = t398.*2.257319383180457e+3;
t606 = t398.*1.744166601788531e+3;
t607 = t398.*3.383303336574349e+3;
t632 = t53+t139+t385;
t633 = t54+t142+t386;
t636 = t262+t398;
t638 = t274+t399;
t646 = -dq5.*(t261-t399);
t647 = -t6.*(t261-t399);
t648 = -t11.*(t261-t399);
t650 = dq5.*(t261-t399);
t651 = -t649;
t662 = t6.*(t261-t399).*(-7.26735103);
t663 = t11.*(t261-t399).*(-7.26735103);
t686 = t6.*(t261-t399).*(-7.263507131821755e+1);
t687 = t11.*(t261-t399).*(-7.263507131821755e+1);
t690 = t6.*(t261-t399).*(-1.336375981993753e+2);
t691 = t11.*(t261-t399).*(-1.336375981993753e+2);
t693 = -t53.*(t261-t399);
t698 = t62.*(t261-t399);
t699 = t6.*(t261-t399).*(-1.40259874879e-5);
t700 = t11.*(t261-t399).*(-1.40259874879e-5);
t722 = t6.*(t261-t399).*(-1.246862890394724e+3);
t723 = t11.*(t261-t399).*(-1.246862890394724e+3);
t726 = t6.*(t261-t399).*(-4.200920957332826e+3);
t727 = t11.*(t261-t399).*(-4.200920957332826e+3);
t729 = t103.*(t261-t399);
t732 = t6.*(t261-t399).*(-3.146556876441599e-4);
t733 = t11.*(t261-t399).*(-3.146556876441599e-4);
t735 = t6.*(t261-t399).*(-4.126305645247942e-4);
t736 = t11.*(t261-t399).*(-4.126305645247942e-4);
t737 = t6.*(t261-t399).*3.146556876441599e-4;
t738 = t11.*(t261-t399).*4.126305645247942e-4;
t743 = t126.*(t261-t399);
t748 = t6.*(t261-t399).*(-3.383303336574349e+3);
t749 = t11.*(t261-t399).*(-1.744166601788531e+3);
t780 = t391.*t612;
t781 = t391.*t615;
t805 = -t804;
t812 = t52+t90+t159+t296+t395;
t813 = t143+t154+t387+t393;
t820 = t119+t397+t635;
t821 = t121+t401+t634;
t856 = t206+t224+t450+t455;
t877 = t5.*t867;
t878 = t10.*t867;
t887 = t225+t238+t456+t480;
t888 = t99+t148+t220+t348+t453;
t889 = t118+t150+t215+t353+t452;
t895 = t104+t147+t239+t350+t481;
t898 = t391.*t811;
t908 = t255.*t855;
t912 = t255.*t892;
t918 = -t883.*(t57+t284);
t919 = t883.*(t57+t284);
t928 = -t896.*(t57+t284);
t937 = -t935;
t939 = t9.*t938;
t940 = t4.*t938;
t941 = t410+t622+t779;
t942 = t29.*t938;
t945 = t61.*t938;
t947 = dq3.*t938.*(-1.705746846438843);
t949 = t4.*t946;
t950 = t9.*t946;
t955 = t5.*t954;
t956 = t10.*t954;
t958 = t12.*t39.*t938.*3.33782865;
t959 = t101.*t938;
t960 = t112.*t938;
t962 = dq3.*t938.*(-1.74926470944712e+1);
t1020 = t363.*t938;
t1028 = t490.*t938;
t1031 = t505.*t938;
t1051 = t628.*t938;
t1063 = t5.*t1062;
t1065 = t10.*t1062.*7.26735103;
t1067 = t10.*t1062.*1.087689656e+1;
t1069 = t10.*t1062.*7.263507131821755e+1;
t1070 = t10.*t1062.*1.336375981993753e+2;
t1072 = t10.*t1062.*6.185536839278779e+1;
t1075 = t10.*t1062.*7.051076542399408e-1;
t1081 = t86+t241+t764+t936;
t407 = -t405;
t472 = t404.*7.26735103;
t473 = t405.*7.26735103;
t528 = t404.*1.336375981993753e+2;
t530 = t405.*1.336375981993753e+2;
t532 = t404.*7.263507131821755e+1;
t533 = t405.*7.263507131821755e+1;
t534 = -t526;
t544 = t404.*1.40259874879e-5;
t545 = t405.*1.40259874879e-5;
t556 = -t550;
t567 = t404.*1.246862890394724e+3;
t568 = t405.*1.246862890394724e+3;
t569 = t404.*4.200920957332826e+3;
t570 = t405.*4.200920957332826e+3;
t580 = -t572;
t588 = t404.*4.126305645247942e-4;
t589 = t405.*4.126305645247942e-4;
t590 = t404.*3.146556876441599e-4;
t591 = t405.*3.146556876441599e-4;
t595 = -t594;
t608 = t404.*1.744166601788531e+3;
t609 = t405.*3.383303336574349e+3;
t637 = dq6+t636;
t640 = dq5.*t636;
t643 = t6.*t636.*6.0;
t644 = t11.*t636.*6.0;
t682 = t650.*(-1.336375981993753e+2);
t683 = t650.*(-7.263507131821755e+1);
t684 = t54.*t636;
t688 = t650.*1.336375981993753e+2;
t689 = t329+t464;
t692 = t342+t466;
t694 = t62.*t636;
t695 = t650.*6.185536839278779e+1;
t697 = t650.*(-7.051076542399408e-1);
t711 = t88.*t636;
t714 = t20+t326+t459;
t719 = t650.*(-7.291450524218959e+2);
t720 = t650.*(-4.200920957332826e+3);
t724 = t100.*t636;
t728 = t650.*(-1.758766552463174e+1);
t730 = t650.*(-4.126305645247942e-4);
t731 = t650.*(-3.146556876441599e-4);
t734 = t650.*4.126305645247942e-4;
t739 = t127.*t636;
t742 = t650.*(-5.878411097842592e+2);
t750 = t373+t525;
t751 = t376+t524;
t752 = t384+t542;
t753 = t388+t537;
t776 = t50+t365+t509;
t778 = t48+t366+t512;
t790 = t400.*t633;
t791 = t400.*t632;
t795 = t404+t648;
t817 = -t48.*(t405+t6.*(t261-t399));
t819 = dq6.*(t405+t6.*(t261-t399)).*(-1.40259874879e-5);
t825 = dq6.*(t405+t6.*(t261-t399)).*(-1.246862890394724e+3);
t828 = dq6.*(t405+t6.*(t261-t399)).*(-3.146556876441599e-4);
t830 = dq6.*(t405+t6.*(t261-t399)).*(-3.383303336574349e+3);
t833 = t10.*t820.*4.234075154e+1;
t839 = t5.*t820.*3.077051043151931e+2;
t840 = t6.*t820.*1.336375981993753e+2;
t842 = t11.*t820.*7.263507131821755e+1;
t843 = t5.*t820.*4.605359747732407e+2;
t844 = t10.*t820.*4.605359747732407e+2;
t849 = t6.*t820.*1.40259874879e-5;
t850 = t11.*t820.*1.40259874879e-5;
t857 = t5.*t820.*5.658316341762099e+3;
t858 = t5.*t820.*3.07542350777483e+3;
t859 = t6.*t820.*1.246862890394724e+3;
t860 = t11.*t820.*1.246862890394724e+3;
t861 = t5.*t820.*2.619002784534197e+3;
t862 = t10.*t820.*5.743628218407764e+3;
t863 = t5.*t820.*2.985478799712556e+1;
t864 = t10.*t820.*2.985478799712556e+1;
t871 = t11.*t820.*4.126305645247942e-4;
t873 = t6.*t820.*3.146556876441599e-4;
t890 = t6.*t820.*3.383303336574349e+3;
t891 = t11.*t820.*1.744166601788531e+3;
t897 = t255.*t813;
t899 = -t812.*(t57+t284);
t900 = t812.*(t57+t284);
t903 = (t261-t399).*(t369-t524);
t904 = t67+t158+t370+t389+t523;
t905 = t62+t153+t378+t394+t526;
t907 = (t261-t399).*(t383-t537);
t909 = -t908;
t913 = -t912;
t914 = t255.*t895;
t917 = t391.*t856;
t920 = t88+t188+t432+t434+t564;
t921 = t391.*t888;
t923 = -t887.*(t57+t284);
t925 = t100+t209+t425+t451+t554;
t926 = t391.*t889;
t927 = t113+t219+t423+t444+t553;
t929 = t128+t235+t440+t465+t571;
t930 = t127+t234+t437+t476+t565;
t931 = t434+t449+t564+t572;
t943 = t33.*t941;
t948 = t122+t650+t823;
t951 = t63.*t941;
t952 = dq3.*t941.*(-2.869063922714997);
t953 = -t950;
t957 = -t956;
t961 = t89+t941;
t963 = t12.*t39.*t941.*3.33782865;
t964 = t105.*t941;
t967 = t111.*t941;
t968 = t949.*2.889644336e+1;
t969 = t950.*2.889644336e+1;
t970 = dq3.*t941.*(-2.942260910305135e+1);
t971 = t949.*1.087689656e+1;
t982 = t949.*6.678442840618982e+2;
t983 = t950.*6.678442840618982e+2;
t984 = t949.*1.356524863046341e+2;
t985 = t950.*1.688943762888624e+2;
t987 = t949.*6.185536839278779e+1;
t997 = t949.*1.870703729528352e-1;
t1021 = t364.*t941;
t1029 = t491.*t941;
t1032 = -t1031;
t1033 = t502.*t941;
t1053 = -t1051;
t1054 = t630.*t941;
t1064 = t362+t803+t878;
t1066 = t1063.*1.087689656e+1;
t1071 = t1063.*1.356524863046341e+2;
t1074 = t1063.*7.051076542399408e-1;
t1082 = t5.*t1081;
t1083 = t10.*t1081;
t1084 = t93+t244+t763+t937;
t1096 = t98+t323+t340+t766+t939;
t1097 = t97+t327+t336+t768+t940;
t1102 = t102+t327+t338+t768+t940;
t1208 = t157+t231+t429+t448+t529+t645+t669+t769+t787+t841+t958;
t477 = -t473;
t538 = -t530;
t540 = -t533;
t546 = -t545;
t575 = -t568;
t576 = -t570;
t592 = -t588;
t593 = -t589;
t611 = -t609;
t696 = t640.*(-7.051076542399408e-1);
t725 = t640.*(-2.524704765397172);
t741 = t640.*(-2.257319383180457e+3);
t792 = -t791;
t798 = t407+t647;
t814 = t472+t663;
t816 = t50.*t795;
t818 = dq6.*t795.*1.40259874879e-5;
t822 = dq6.*t795.*1.246862890394724e+3;
t826 = dq6.*t795.*4.126305645247942e-4;
t827 = -t116.*t795;
t829 = dq6.*t795.*1.744166601788531e+3;
t831 = t528+t691;
t834 = -t833;
t835 = t544+t700;
t874 = -t871;
t901 = t636.*t750;
t906 = t636.*t752;
t910 = t637.*t776;
t911 = t637.*t778;
t915 = -t914;
t916 = t370+t371+t523+t534;
t922 = t88+t188+t432+t439+t580;
t924 = -t921;
t932 = t420+t461+t549+t595;
t933 = t419+t467+t556+t596;
t944 = t123+t640+t824;
h = ft_2({dq1,dq2,dq3,dq4,dq5,dq6,t10,t1020,t1021,t1028,t1029,t1032,t1033,t104,t1051,t1053,t1054,t106,t1062,t1063,t1064,t1065,t1066,t1067,t1069,t1070,t1071,t1072,t1074,t1075,t1081,t1082,t1083,t1096,t1097,t11,t1102,t116,t117,t12,t120,t1208,t13,t130,t131,t134,t136,t141,t149,t155,t156,t169,t170,t174,t178,t191,t194,t196,t197,t198,t2,t20,t201,t202,t203,t204,t205,t207,t208,t210,t211,t212,t216,t217,t218,t222,t223,t226,t228,t229,t23,t232,t244,t254,t256,t257,t258,t259,t261,t264,t266,t267,t268,t269,t270,t276,t277,t278,t28,t280,t281,t282,t283,t284,t285,t286,t287,t288,t289,t291,t292,t293,t294,t295,t3,t302,t303,t305,t308,t309,t311,t314,t328,t331,t333,t337,t34,t349,t359,t360,t362,t369,t374,t383,t39,t390,t392,t397,t399,t4,t40,t400,t405,t408,t415,t416,t417,t418,t421,t430,t435,t436,t443,t447,t45,t457,t466,t468,t471,t473,t474,t475,t477,t48,t482,t483,t485,t486,t487,t488,t489,t49,t493,t495,t496,t497,t499,t5,t50,t501,t504,t506,t507,t508,t510,t511,t514,t515,t516,t517,t518,t52,t520,t521,t522,t524,t527,t53,t530,t532,t533,t537,t538,t539,t54,t540,t541,t543,t545,t546,t547,t548,t55,t552,t555,t557,t558,t56,t560,t561,t562,t563,t566,t567,t568,t569,t57,t574,t575,t576,t577,t578,t579,t58,t581,t582,t583,t585,t586,t587,t588,t590,t591,t592,t593,t597,t598,t6,t60,t601,t603,t604,t605,t606,t607,t608,t609,t610,t611,t612,t615,t62,t621,t625,t626,t629,t632,t633,t636,t637,t640,t642,t643,t644,t65,t650,t651,t652,t653,t655,t658,t659,t66,t661,t662,t664,t666,t667,t668,t670,t671,t672,t673,t674,t675,t676,t678,t679,t68,t680,t681,t683,t684,t685,t686,t687,t688,t689,t690,t693,t695,t696,t698,t699,t7,t705,t706,t707,t709,t710,t711,t712,t714,t715,t717,t718,t719,t72,t720,t721,t722,t723,t725,t726,t727,t729,t73,t731,t733,t734,t735,t736,t737,t738,t74,t740,t741,t743,t744,t747,t748,t749,t75,t750,t752,t754,t756,t757,t758,t76,t760,t761,t762,t763,t765,t77,t770,t772,t773,t775,t776,t778,t78,t780,t781,t782,t783,t786,t789,t79,t790,t792,t793,t794,t795,t796,t797,t799,t8,t80,t800,t801,t802,t805,t806,t807,t808,t809,t81,t810,t811,t812,t813,t814,t816,t817,t818,t819,t820,t822,t825,t826,t827,t828,t829,t830,t831,t833,t834,t835,t837,t839,t84,t840,t842,t843,t844,t845,t847,t848,t849,t85,t850,t851,t852,t854,t857,t858,t859,t860,t861,t862,t863,t864,t866,t867,t868,t869,t870,t871,t872,t873,t874,t876,t877,t879,t880,t882,t884,t886,t887,t890,t891,t894,t897,t898,t899,t9,t900,t901,t903,t904,t905,t906,t907,t908,t909,t91,t910,t911,t913,t915,t916,t917,t919,t92,t920,t922,t923,t924,t925,t926,t927,t928,t929,t930,t931,t932,t933,t934,t935,t938,t941,t942,t943,t947,t948,t949,t950,t952,t953,t954,t955,t957,t959,t96,t960,t961,t962,t963,t964,t967,t968,t969,t970,t971,t982,t983,t984,t985,t987,t997});
end
function h = ft_2(ct)
dq1 = ct{1};
dq2 = ct{2};
dq3 = ct{3};
dq4 = ct{4};
dq5 = ct{5};
dq6 = ct{6};
t10 = ct{7};
t1020 = ct{8};
t1021 = ct{9};
t1028 = ct{10};
t1029 = ct{11};
t1032 = ct{12};
t1033 = ct{13};
t104 = ct{14};
t1051 = ct{15};
t1053 = ct{16};
t1054 = ct{17};
t106 = ct{18};
t1062 = ct{19};
t1063 = ct{20};
t1064 = ct{21};
t1065 = ct{22};
t1066 = ct{23};
t1067 = ct{24};
t1069 = ct{25};
t1070 = ct{26};
t1071 = ct{27};
t1072 = ct{28};
t1074 = ct{29};
t1075 = ct{30};
t1081 = ct{31};
t1082 = ct{32};
t1083 = ct{33};
t1096 = ct{34};
t1097 = ct{35};
t11 = ct{36};
t1102 = ct{37};
t116 = ct{38};
t117 = ct{39};
t12 = ct{40};
t120 = ct{41};
t1208 = ct{42};
t13 = ct{43};
t130 = ct{44};
t131 = ct{45};
t134 = ct{46};
t136 = ct{47};
t141 = ct{48};
t149 = ct{49};
t155 = ct{50};
t156 = ct{51};
t169 = ct{52};
t170 = ct{53};
t174 = ct{54};
t178 = ct{55};
t191 = ct{56};
t194 = ct{57};
t196 = ct{58};
t197 = ct{59};
t198 = ct{60};
t2 = ct{61};
t20 = ct{62};
t201 = ct{63};
t202 = ct{64};
t203 = ct{65};
t204 = ct{66};
t205 = ct{67};
t207 = ct{68};
t208 = ct{69};
t210 = ct{70};
t211 = ct{71};
t212 = ct{72};
t216 = ct{73};
t217 = ct{74};
t218 = ct{75};
t222 = ct{76};
t223 = ct{77};
t226 = ct{78};
t228 = ct{79};
t229 = ct{80};
t23 = ct{81};
t232 = ct{82};
t244 = ct{83};
t254 = ct{84};
t256 = ct{85};
t257 = ct{86};
t258 = ct{87};
t259 = ct{88};
t261 = ct{89};
t264 = ct{90};
t266 = ct{91};
t267 = ct{92};
t268 = ct{93};
t269 = ct{94};
t270 = ct{95};
t276 = ct{96};
t277 = ct{97};
t278 = ct{98};
t28 = ct{99};
t280 = ct{100};
t281 = ct{101};
t282 = ct{102};
t283 = ct{103};
t284 = ct{104};
t285 = ct{105};
t286 = ct{106};
t287 = ct{107};
t288 = ct{108};
t289 = ct{109};
t291 = ct{110};
t292 = ct{111};
t293 = ct{112};
t294 = ct{113};
t295 = ct{114};
t3 = ct{115};
t302 = ct{116};
t303 = ct{117};
t305 = ct{118};
t308 = ct{119};
t309 = ct{120};
t311 = ct{121};
t314 = ct{122};
t328 = ct{123};
t331 = ct{124};
t333 = ct{125};
t337 = ct{126};
t34 = ct{127};
t349 = ct{128};
t359 = ct{129};
t360 = ct{130};
t362 = ct{131};
t369 = ct{132};
t374 = ct{133};
t383 = ct{134};
t39 = ct{135};
t390 = ct{136};
t392 = ct{137};
t397 = ct{138};
t399 = ct{139};
t4 = ct{140};
t40 = ct{141};
t400 = ct{142};
t405 = ct{143};
t408 = ct{144};
t415 = ct{145};
t416 = ct{146};
t417 = ct{147};
t418 = ct{148};
t421 = ct{149};
t430 = ct{150};
t435 = ct{151};
t436 = ct{152};
t443 = ct{153};
t447 = ct{154};
t45 = ct{155};
t457 = ct{156};
t466 = ct{157};
t468 = ct{158};
t471 = ct{159};
t473 = ct{160};
t474 = ct{161};
t475 = ct{162};
t477 = ct{163};
t48 = ct{164};
t482 = ct{165};
t483 = ct{166};
t485 = ct{167};
t486 = ct{168};
t487 = ct{169};
t488 = ct{170};
t489 = ct{171};
t49 = ct{172};
t493 = ct{173};
t495 = ct{174};
t496 = ct{175};
t497 = ct{176};
t499 = ct{177};
t5 = ct{178};
t50 = ct{179};
t501 = ct{180};
t504 = ct{181};
t506 = ct{182};
t507 = ct{183};
t508 = ct{184};
t510 = ct{185};
t511 = ct{186};
t514 = ct{187};
t515 = ct{188};
t516 = ct{189};
t517 = ct{190};
t518 = ct{191};
t52 = ct{192};
t520 = ct{193};
t521 = ct{194};
t522 = ct{195};
t524 = ct{196};
t527 = ct{197};
t53 = ct{198};
t530 = ct{199};
t532 = ct{200};
t533 = ct{201};
t537 = ct{202};
t538 = ct{203};
t539 = ct{204};
t54 = ct{205};
t540 = ct{206};
t541 = ct{207};
t543 = ct{208};
t545 = ct{209};
t546 = ct{210};
t547 = ct{211};
t548 = ct{212};
t55 = ct{213};
t552 = ct{214};
t555 = ct{215};
t557 = ct{216};
t558 = ct{217};
t56 = ct{218};
t560 = ct{219};
t561 = ct{220};
t562 = ct{221};
t563 = ct{222};
t566 = ct{223};
t567 = ct{224};
t568 = ct{225};
t569 = ct{226};
t57 = ct{227};
t574 = ct{228};
t575 = ct{229};
t576 = ct{230};
t577 = ct{231};
t578 = ct{232};
t579 = ct{233};
t58 = ct{234};
t581 = ct{235};
t582 = ct{236};
t583 = ct{237};
t585 = ct{238};
t586 = ct{239};
t587 = ct{240};
t588 = ct{241};
t590 = ct{242};
t591 = ct{243};
t592 = ct{244};
t593 = ct{245};
t597 = ct{246};
t598 = ct{247};
t6 = ct{248};
t60 = ct{249};
t601 = ct{250};
t603 = ct{251};
t604 = ct{252};
t605 = ct{253};
t606 = ct{254};
t607 = ct{255};
t608 = ct{256};
t609 = ct{257};
t610 = ct{258};
t611 = ct{259};
t612 = ct{260};
t615 = ct{261};
t62 = ct{262};
t621 = ct{263};
t625 = ct{264};
t626 = ct{265};
t629 = ct{266};
t632 = ct{267};
t633 = ct{268};
t636 = ct{269};
t637 = ct{270};
t640 = ct{271};
t642 = ct{272};
t643 = ct{273};
t644 = ct{274};
t65 = ct{275};
t650 = ct{276};
t651 = ct{277};
t652 = ct{278};
t653 = ct{279};
t655 = ct{280};
t658 = ct{281};
t659 = ct{282};
t66 = ct{283};
t661 = ct{284};
t662 = ct{285};
t664 = ct{286};
t666 = ct{287};
t667 = ct{288};
t668 = ct{289};
t670 = ct{290};
t671 = ct{291};
t672 = ct{292};
t673 = ct{293};
t674 = ct{294};
t675 = ct{295};
t676 = ct{296};
t678 = ct{297};
t679 = ct{298};
t68 = ct{299};
t680 = ct{300};
t681 = ct{301};
t683 = ct{302};
t684 = ct{303};
t685 = ct{304};
t686 = ct{305};
t687 = ct{306};
t688 = ct{307};
t689 = ct{308};
t690 = ct{309};
t693 = ct{310};
t695 = ct{311};
t696 = ct{312};
t698 = ct{313};
t699 = ct{314};
t7 = ct{315};
t705 = ct{316};
t706 = ct{317};
t707 = ct{318};
t709 = ct{319};
t710 = ct{320};
t711 = ct{321};
t712 = ct{322};
t714 = ct{323};
t715 = ct{324};
t717 = ct{325};
t718 = ct{326};
t719 = ct{327};
t72 = ct{328};
t720 = ct{329};
t721 = ct{330};
t722 = ct{331};
t723 = ct{332};
t725 = ct{333};
t726 = ct{334};
t727 = ct{335};
t729 = ct{336};
t73 = ct{337};
t731 = ct{338};
t733 = ct{339};
t734 = ct{340};
t735 = ct{341};
t736 = ct{342};
t737 = ct{343};
t738 = ct{344};
t74 = ct{345};
t740 = ct{346};
t741 = ct{347};
t743 = ct{348};
t744 = ct{349};
t747 = ct{350};
t748 = ct{351};
t749 = ct{352};
t75 = ct{353};
t750 = ct{354};
t752 = ct{355};
t754 = ct{356};
t756 = ct{357};
t757 = ct{358};
t758 = ct{359};
t76 = ct{360};
t760 = ct{361};
t761 = ct{362};
t762 = ct{363};
t763 = ct{364};
t765 = ct{365};
t77 = ct{366};
t770 = ct{367};
t772 = ct{368};
t773 = ct{369};
t775 = ct{370};
t776 = ct{371};
t778 = ct{372};
t78 = ct{373};
t780 = ct{374};
t781 = ct{375};
t782 = ct{376};
t783 = ct{377};
t786 = ct{378};
t789 = ct{379};
t79 = ct{380};
t790 = ct{381};
t792 = ct{382};
t793 = ct{383};
t794 = ct{384};
t795 = ct{385};
t796 = ct{386};
t797 = ct{387};
t799 = ct{388};
t8 = ct{389};
t80 = ct{390};
t800 = ct{391};
t801 = ct{392};
t802 = ct{393};
t805 = ct{394};
t806 = ct{395};
t807 = ct{396};
t808 = ct{397};
t809 = ct{398};
t81 = ct{399};
t810 = ct{400};
t811 = ct{401};
t812 = ct{402};
t813 = ct{403};
t814 = ct{404};
t816 = ct{405};
t817 = ct{406};
t818 = ct{407};
t819 = ct{408};
t820 = ct{409};
t822 = ct{410};
t825 = ct{411};
t826 = ct{412};
t827 = ct{413};
t828 = ct{414};
t829 = ct{415};
t830 = ct{416};
t831 = ct{417};
t833 = ct{418};
t834 = ct{419};
t835 = ct{420};
t837 = ct{421};
t839 = ct{422};
t84 = ct{423};
t840 = ct{424};
t842 = ct{425};
t843 = ct{426};
t844 = ct{427};
t845 = ct{428};
t847 = ct{429};
t848 = ct{430};
t849 = ct{431};
t85 = ct{432};
t850 = ct{433};
t851 = ct{434};
t852 = ct{435};
t854 = ct{436};
t857 = ct{437};
t858 = ct{438};
t859 = ct{439};
t860 = ct{440};
t861 = ct{441};
t862 = ct{442};
t863 = ct{443};
t864 = ct{444};
t866 = ct{445};
t867 = ct{446};
t868 = ct{447};
t869 = ct{448};
t870 = ct{449};
t871 = ct{450};
t872 = ct{451};
t873 = ct{452};
t874 = ct{453};
t876 = ct{454};
t877 = ct{455};
t879 = ct{456};
t880 = ct{457};
t882 = ct{458};
t884 = ct{459};
t886 = ct{460};
t887 = ct{461};
t890 = ct{462};
t891 = ct{463};
t894 = ct{464};
t897 = ct{465};
t898 = ct{466};
t899 = ct{467};
t9 = ct{468};
t900 = ct{469};
t901 = ct{470};
t903 = ct{471};
t904 = ct{472};
t905 = ct{473};
t906 = ct{474};
t907 = ct{475};
t908 = ct{476};
t909 = ct{477};
t91 = ct{478};
t910 = ct{479};
t911 = ct{480};
t913 = ct{481};
t915 = ct{482};
t916 = ct{483};
t917 = ct{484};
t919 = ct{485};
t92 = ct{486};
t920 = ct{487};
t922 = ct{488};
t923 = ct{489};
t924 = ct{490};
t925 = ct{491};
t926 = ct{492};
t927 = ct{493};
t928 = ct{494};
t929 = ct{495};
t930 = ct{496};
t931 = ct{497};
t932 = ct{498};
t933 = ct{499};
t934 = ct{500};
t935 = ct{501};
t938 = ct{502};
t941 = ct{503};
t942 = ct{504};
t943 = ct{505};
t947 = ct{506};
t948 = ct{507};
t949 = ct{508};
t950 = ct{509};
t952 = ct{510};
t953 = ct{511};
t954 = ct{512};
t955 = ct{513};
t957 = ct{514};
t959 = ct{515};
t96 = ct{516};
t960 = ct{517};
t961 = ct{518};
t962 = ct{519};
t963 = ct{520};
t964 = ct{521};
t967 = ct{522};
t968 = ct{523};
t969 = ct{524};
t970 = ct{525};
t971 = ct{526};
t982 = ct{527};
t983 = ct{528};
t984 = ct{529};
t985 = ct{530};
t987 = ct{531};
t997 = ct{532};
t965 = t5.*t961;
t966 = t10.*t961;
t972 = -t968;
t973 = t6.*t948.*4.360410618e+1;
t974 = t11.*t948.*4.360410618e+1;
t976 = -t971;
t979 = t6.*(t120-t640+t10.*(dq4.*(t57+t284)+dq3.*t57.*5.110348748545983e-1+t4.*(t328-t331))).*(-7.263507131821755e+1);
t980 = t11.*(t120-t640+t10.*(dq4.*(t57+t284)+dq3.*t57.*5.110348748545983e-1+t4.*(t328-t331))).*(-1.336375981993753e+2);
t981 = t6.*(t120-t640+t10.*(dq4.*(t57+t284)+dq3.*t57.*5.110348748545983e-1+t4.*(t328-t331))).*7.263507131821755e+1;
t986 = -t983;
t988 = t11.*t948.*4.358104279093053e+2;
t989 = -t985;
t990 = t6.*t948.*8.018255891962515e+2;
t991 = -t987;
t994 = t6.*(t120-t640+t10.*(dq4.*(t57+t284)+dq3.*t57.*5.110348748545983e-1+t4.*(t328-t331))).*(-1.40259874879e-5);
t995 = t11.*(t120-t640+t10.*(dq4.*(t57+t284)+dq3.*t57.*5.110348748545983e-1+t4.*(t328-t331))).*(-1.40259874879e-5);
t996 = t6.*(t120-t640+t10.*(dq4.*(t57+t284)+dq3.*t57.*5.110348748545983e-1+t4.*(t328-t331))).*1.40259874879e-5;
t998 = t400.*t925;
t999 = -t997;
t1000 = t6.*t948.*8.415592492740001e-5;
t1001 = t11.*t948.*8.415592492740001e-5;
t1004 = t400.*t927;
t1006 = t6.*(t120-t640+t10.*(dq4.*(t57+t284)+dq3.*t57.*5.110348748545983e-1+t4.*(t328-t331))).*(-1.246862890394724e+3);
t1007 = t11.*(t120-t640+t10.*(dq4.*(t57+t284)+dq3.*t57.*5.110348748545983e-1+t4.*(t328-t331))).*(-1.246862890394724e+3);
t1008 = t6.*(t120-t640+t10.*(dq4.*(t57+t284)+dq3.*t57.*5.110348748545983e-1+t4.*(t328-t331))).*1.246862890394724e+3;
t1009 = t11.*(t120-t640+t10.*(dq4.*(t57+t284)+dq3.*t57.*5.110348748545983e-1+t4.*(t328-t331))).*(-3.146556876441599e-4);
t1010 = t6.*(t120-t640+t10.*(dq4.*(t57+t284)+dq3.*t57.*5.110348748545983e-1+t4.*(t328-t331))).*(-4.126305645247942e-4);
t1011 = t636.*t905;
t1012 = -t904.*(t261-t399);
t1013 = t904.*(t261-t399);
t1014 = t6.*(t120-t640+t10.*(dq4.*(t57+t284)+dq3.*t57.*5.110348748545983e-1+t4.*(t328-t331))).*(-1.744166601788531e+3);
t1015 = t11.*(t120-t640+t10.*(dq4.*(t57+t284)+dq3.*t57.*5.110348748545983e-1+t4.*(t328-t331))).*(-3.383303336574349e+3);
t1016 = t6.*(t120-t640+t10.*(dq4.*(t57+t284)+dq3.*t57.*5.110348748545983e-1+t4.*(t328-t331))).*1.744166601788531e+3;
t1017 = t66+t390+t532+t543+t687;
t1019 = t400.*t931;
t1023 = (t533+t6.*(t261-t399).*7.263507131821755e+1).*(t405+t6.*(t261-t399));
t1026 = (t405+t6.*(t261-t399)).*(t545+t6.*(t261-t399).*1.40259874879e-5);
t1030 = -t1029;
t1034 = -t920.*(t261-t399);
t1036 = t84+t421+t552+t591+t737;
t1038 = t117+t447+t569+t578+t727;
t1040 = t636.*t929;
t1042 = -t930.*(t261-t399);
t1044 = t131+t487+t590+t607+t733;
t1046 = t510.*t961;
t1047 = -t961.*(t96-t333);
t1055 = -t1054;
t1056 = t604.*t961;
t1058 = t610.*t961;
t1059 = t588+t591+t736+t737;
t1068 = -t1066;
t1073 = -t1071;
t1076 = -t1074;
t1079 = -t637.*(t530-t532+t6.*(t261-t399).*1.336375981993753e+2+t11.*(t261-t399).*7.263507131821755e+1);
t1080 = t813.*t961;
t1098 = dq4.*t1096;
t1099 = t5.*t1096;
t1100 = t10.*t1096;
t1101 = dq4.*t1097;
t1104 = t6.*t1102;
t1105 = t11.*t1102;
t1106 = t23.*t1096;
t1110 = t23.*t1097;
t1112 = t52.*t1096;
t1116 = t52.*t1097;
t1117 = t56.*t1097;
t1118 = t65.*t1096;
et1 = -t567+t609+t6.*(t261-t399).*3.383303336574349e+3;
et2 = t11.*(t261-t399).*1.246862890394724e+3;
t1120 = -t795.*(et1+et2);
et3 = t568-t608+t6.*(t261-t399).*1.246862890394724e+3;
et4 = t11.*(t261-t399).*1.744166601788531e+3;
t1121 = (et3+et4).*(t405+t6.*(t261-t399));
t1123 = t417.*t1096;
t1124 = t417.*t1097;
t1125 = -t1096.*(t96-t333);
t1126 = t510.*t1097;
t1127 = t1096.*(t96-t333);
t1128 = t612.*t1096;
t1129 = t615.*t1096;
t1131 = -t1097.*(t134-t374);
t1132 = t1097.*(t134-t374);
t1133 = -t1097.*(t156-t392);
t1134 = t1097.*(t156-t392);
t1135 = t632.*t1102;
t1136 = t633.*t1102;
t1137 = t689.*t1102;
t1138 = -t1102.*(t337-t466);
t1140 = t349+t359+t942+t943;
t1149 = t811.*t1096;
t1151 = t812.*t1097;
t1163 = t362+t955+t1083;
t1209 = t155+t232+t435+t436+t517+t651+t668+t772+t789+t837+t963;
t1242 = t212+t415+t416+t605+t670+t671+t947+t952+t1020+t1021;
t1257 = t288+t495+t499+t557+t560+t629+t659+t661+t760+t761+t794+t894+t1032+t1033;
et5 = t305+t482-t488+t504+t577-t667-t757-t800-t808+t809+t960+t964-t1028+t1054-dq3.*t257.*2.65855123043135e-4;
et6 = dq3.*t765.*(-8.818711196088817e-6);
t1264 = t34.*t40.*(et5+et6).*(-9.543032792050485e-17);
et7 = t305+t482-t488+t504+t577-t667-t757-t800-t808+t809+t960+t964-t1028+t1054-dq3.*t257.*2.65855123043135e-4;
et8 = dq3.*t765.*(-8.818711196088817e-6);
t1265 = t34.*t40.*(et7+et8).*9.543032792050485e-17;
t815 = t477+t662;
t832 = t540+t686;
t836 = t546+t699;
t902 = -t901;
t975 = -t966;
t977 = -t974;
t978 = t400.*t916;
t992 = -t988;
t993 = -t990;
t1002 = -t998;
t1003 = -t1001;
t1005 = -t1004;
t1018 = t66+t390+t538+t543+t690;
t1022 = t795.*t831;
t1024 = t795.*t835;
t1027 = -t1026;
t1035 = t636.*t922;
t1037 = t84+t421+t552+t592+t738;
t1039 = t116+t443+t576+t582+t726;
t1041 = -t1040;
t1043 = t532+t538+t687+t690;
t1045 = t130+t486+t593+t606+t735;
t1048 = t636.*t932;
t1050 = -t933.*(t261-t399);
t1052 = t933.*(t261-t399);
t1057 = -t1056;
t1060 = t575+t608+t722+t749;
t1061 = t567+t611+t723+t748;
t1077 = t637.*t1038;
t1086 = -t1017.*(t405+t6.*(t261-t399));
t1088 = t1017.*(t405+t6.*(t261-t399));
t1089 = t637.*t1059;
t1090 = t795.*t1036;
t1092 = t795.*t1044;
t1103 = -t1099;
t1107 = t1098.*1.087689656e+1;
t1108 = t1098.*(-2.889644336e+1);
t1111 = t1101.*(-2.889644336e+1);
t1113 = t1098.*6.185536839278779e+1;
t1114 = t1098.*1.356524863046341e+2;
t1119 = t1098.*(-1.870703729528352e-1);
t1122 = -t1121;
t1130 = -t1128;
t1139 = -t1137;
t1141 = t4.*t1140;
t1142 = t9.*t1140;
t1150 = -t1149;
t1152 = -t1151;
t1161 = t916.*t1102;
t1164 = t475+t965+t1100;
t1258 = t39.*t1257;
t1260 = t203+t226+t418+t430+t515+t539+t541+t642+t680+t685+t780+t782+t786+t897+t1126+t1127;
t1261 = t303+t483+t489+t506+t507+t585+t666+t758+t797+t801+t806+t807+t959+t967+t1030+t1053;
t1262 = t309+t485+t488+t508+t514+t583+t667+t757+t799+t800+t808+t810+t962+t970+t1028+t1055;
t1025 = -t1024;
t1049 = -t1048;
t1078 = t637.*t1039;
t1085 = t795.*t1018;
t1091 = -t1037.*(t405+t6.*(t261-t399));
t1093 = -t1092;
t1094 = -t1045.*(t405+t6.*(t261-t399));
t1095 = t1045.*(t405+t6.*(t261-t399));
t1109 = -t1107;
t1115 = -t1113;
t1143 = t1141.*2.889644336e+1;
t1144 = t1142.*2.889644336e+1;
t1145 = t1142.*1.087689656e+1;
t1153 = t1141.*6.678442840618982e+2;
t1154 = t1142.*6.678442840618982e+2;
t1155 = t1141.*1.688943762888624e+2;
t1156 = t1142.*1.356524863046341e+2;
t1157 = t1142.*6.185536839278779e+1;
t1159 = t1142.*1.870703729528352e-1;
t1162 = -t1161;
t1165 = t468+t966+t1103;
t1166 = t6.*t1164;
t1167 = t11.*t1164;
t1168 = -dq5.*(t474+t975+t1099);
t1170 = dq5.*t1164.*7.26735103;
t1172 = t28.*t1164;
t1173 = -t28.*(t474+t975+t1099);
t1174 = dq5.*t1164.*(-1.087689656e+1);
t1175 = dq5.*(t474+t975+t1099).*1.087689656e+1;
t1176 = dq5.*t1164.*1.336375981993753e+2;
t1177 = dq5.*t1164.*7.263507131821755e+1;
t1180 = t53.*t1164;
t1181 = dq5.*t1164.*(-6.185536839278779e+1);
t1182 = dq5.*(t474+t975+t1099).*(-1.356524863046341e+2);
t1183 = t62.*t1164;
t1184 = t54.*(t474+t975+t1099);
t1185 = dq5.*(t474+t975+t1099).*(-7.051076542399408e-1);
t1186 = dq5.*t1164.*(-7.051076542399408e-1);
t1187 = t62.*(t474+t975+t1099);
t1188 = t13+t60+t285+t474+t975+t1099;
t1189 = t586.*t1164;
t1190 = -t586.*(t474+t975+t1099);
t1191 = t689.*t1164;
t1192 = (t337-t466).*(t474+t975+t1099);
t1193 = -t750.*(t474+t975+t1099);
t1194 = -t1164.*(t369-t524);
t1195 = t1164.*(t369-t524);
t1196 = -t752.*(t474+t975+t1099);
t1197 = -t1164.*(t383-t537);
t1198 = t752.*(t474+t975+t1099);
t1202 = t904.*t1164;
t1203 = -t905.*(t474+t975+t1099);
t1224 = t136+t653+t953+t1101+t1141;
t1240 = t149+t471+t655+t949+t1098+t1142;
t1259 = -t1258;
t1263 = t34.*t40.*t1261.*5.673626844500105e-17;
t1087 = -t1085;
t1146 = -t1143;
t1147 = -t1144;
t1148 = -t1145;
t1158 = -t1157;
t1160 = -t1159;
t1169 = -t1167;
t1171 = -t1170;
t1178 = -t1176;
t1179 = -t1177;
t1199 = t776.*t1188;
t1200 = t778.*t1188;
t1204 = -t1202;
t1205 = t814.*t1188;
t1206 = -t1188.*(t473+t6.*(t261-t399).*7.26735103);
t1207 = t1188.*(t473+t6.*(t261-t399).*7.26735103);
t1210 = -t1188.*(t530-t532+t6.*(t261-t399).*1.336375981993753e+2+t11.*(t261-t399).*7.263507131821755e+1);
t1211 = t644+t1105+t1166;
t1225 = t10.*t1224;
t1229 = t5.*t1224.*7.26735103;
t1230 = t5.*t1224.*1.087689656e+1;
t1232 = t5.*t1224.*7.263507131821755e+1;
t1233 = t5.*t1224.*1.336375981993753e+2;
t1235 = t5.*t1224.*6.185536839278779e+1;
t1236 = t5.*t1224.*7.051076542399408e-1;
t1244 = t6.*t1240.*7.26735103;
t1245 = t11.*t1240.*7.26735103;
t1250 = t6.*t1240.*1.336375981993753e+2;
t1251 = t11.*t1240.*7.263507131821755e+1;
t1252 = t6.*t1240.*1.40259874879e-5;
t1253 = t11.*t1240.*1.40259874879e-5;
t1276 = t276+t277+t282+t493+t496+t555+t574+t581+t658+t717+t718+t793+t913+t926+t928+t982+t1058+t1112+t1134+t1150+t1154;
t1277 = t256+t283+t295+t497+t501+t566+t587+t597+t664+t721+t740+t796+t915+t919+t924+t986+t1057+t1116+t1129+t1152+t1153;
et9 = -t270-t286-t294-t397.*6.597219446016286e+2+t908-t917+t985+t997-t1080-t1101.*1.688943762888624e+2+t1118+t1128+t1131-t1155+t1159+t104.*(t57+t284);
et10 = t887.*(t57+t284)+t4.*(t328-t331).*9.245169992678717;
et11 = t9.*(t328-t331).*4.522154679359383e+3;
t1285 = t34.*t40.*(et9+et10+et11).*(-9.543032792050485e-17);
t1201 = -t1200;
t1212 = t643+t1104+t1169;
t1213 = t20.*t1211;
t1214 = dq6.*t1211.*(-7.26735103);
t1217 = t48.*t1211;
t1220 = t66.*t1211;
t1221 = dq6.*t1211.*(-1.40259874879e-5);
t1226 = -t1225;
t1227 = t714.*t1211;
t1231 = t1225.*1.087689656e+1;
t1234 = t1225.*1.356524863046341e+2;
t1237 = t1225.*7.051076542399408e-1;
t1238 = t814.*t1211;
t1241 = -t1211.*(t533+t6.*(t261-t399).*7.263507131821755e+1);
t1246 = -t1244;
t1247 = -t1211.*(t545+t6.*(t261-t399).*1.40259874879e-5);
t1249 = t1211.*(t545+t6.*(t261-t399).*1.40259874879e-5);
t1254 = -t1252;
t1255 = t1017.*t1211;
t1267 = t6.*(t833-t1063+t1225+dq5.*(t474+t975+t1099)).*(-7.26735103);
t1268 = t11.*(t833-t1063+t1225+dq5.*(t474+t975+t1099)).*(-7.26735103);
t1269 = t11.*(t833-t1063+t1225+dq5.*(t474+t975+t1099)).*(-1.336375981993753e+2);
t1270 = t6.*(t833-t1063+t1225+dq5.*(t474+t975+t1099)).*(-7.263507131821755e+1);
t1271 = t11.*(t833-t1063+t1225+dq5.*(t474+t975+t1099)).*1.336375981993753e+2;
t1272 = t6.*(t833-t1063+t1225+dq5.*(t474+t975+t1099)).*(-1.40259874879e-5);
t1273 = t11.*(t833-t1063+t1225+dq5.*(t474+t975+t1099)).*(-1.40259874879e-5);
t1274 = t218+t222+t527+t673+t744+t781+t900+t972+t1046+t1108+t1123+t1147;
t1275 = t204+t217+t521+t676+t747+t783+t898+t969+t1047+t1111+t1124+t1146;
t1278 = t308.*t1276;
t1280 = t302.*t1277;
t1281 = t202+t205+t223+t522+t681+t684+t695+t848+t851+t906+t907+t976+t978+t1109+t1148+t1191+t1192;
t1282 = t207+t228+t518+t679+t696+t790+t843+t854+t903+t1011+t1067+t1138+t1174+t1189+t1230;
t1284 = t270+t286+t294+t548+t579+t705+t712+t909+t917+t923+t989+t999+t1080+t1117+t1119+t1130+t1132+t1155+t1160;
t1287 = t259+t269+t281+t292+t561+t562+t709+t710+t719+t741+t863+t869+t886+t984+t1005+t1034+t1041+t1075+t1114+t1135+t1156+t1186+t1193+t1204+t1236;
t1215 = t20.*t1212;
t1216 = dq6.*t1212.*(-7.26735103);
t1218 = t50.*t1212;
t1219 = dq6.*t1212.*(-7.263507131821755e+1);
t1222 = t66.*t1212;
t1223 = dq6.*t1212.*(-1.40259874879e-5);
t1228 = t714.*t1212;
t1239 = -t1212.*(t473+t6.*(t261-t399).*7.26735103);
t1243 = t831.*t1212;
t1248 = t835.*t1212;
t1256 = t1018.*t1212;
t1266 = t834+t1063+t1168+t1226;
t1279 = -t1278;
t1283 = t208+t229+t520+t678+t698+t792+t844+t852+t902+t1013+t1068+t1139+t1175+t1190+t1231;
t1288 = t266+t267+t280+t293+t558+t563+t707+t711+t715+t743+t864+t866+t884+t991+t1002+t1035+t1042+t1076+t1115+t1136+t1158+t1187+t1195+t1203+t1237;
t1289 = -t1287.*(t174-t314);
et12 = t266+t267+t280+t293+t558+t563+t640.*7.291450524218959e+2;
et13 = t650.*5.878411097842592e+2+t707+t715+t864+t866+t884+t991+t1002+t1035+t1042+t1076+t1115+t1136+t1158+t1195+t1203+t1237+dq5.*(t474+t975+t1099).*7.051076542399408e-1;
t1290 = t598.*(et12+et13);
t1291 = t1287.*(t174-t314);
t1292 = t258+t278+t287+t547+t706+t725+t729+t861+t862+t876+t879+t1019+t1049+t1052+t1072+t1073+t1162+t1181+t1184+t1197+t1198+t1234+t1235;
t1294 = t198+t688+t818+t845+t850+t910+t973+t996+t1023+t1087+t1207+t1214+t1227+t1246+t1268;
t1286 = t141+t457+t652+t816+t817+t839+t840+t842+t980+t981+t1025+t1027+t1065+t1079+t1171+t1229+t1238+t1239;
t1293 = t302.*t1292;
t1295 = t201+t683+t819+t847+t849+t911+t977+t995+t1022+t1088+t1205+t1216+t1228+t1245+t1267;
t1296 = t194+t289+t511+t672+t734+t825+t829+t858+t859+t880+t891+t1000+t1007+t1016+t1069+t1077+t1091+t1093+t1179+t1201+t1221+t1232+t1243+t1254+t1255+t1273;
t1297 = t191+t291+t516+t675+t731+t822+t830+t857+t860+t882+t890+t1003+t1008+t1015+t1070+t1078+t1090+t1095+t1178+t1199+t1223+t1233+t1241+t1253+t1256+t1272;
t1301 = t268+t720+t827+t828+t870+t873+t874+t992+t993+t1009+t1010+t1089+t1120+t1122+t1210+t1217+t1219+t1248+t1249+t1250+t1251+t1270+t1271;
et14 = -t567+t609+t6.*(t261-t399).*3.383303336574349e+3;
et15 = t11.*(t261-t399).*1.246862890394724e+3;
et16 = t264+t650.*4.200920957332826e+3+t826+t868+t871-t873+t988+t990-t1089+t1121-t1217+t1247-t1248-t1250-t1251+t1269+t795.*(et14+et15)+t117.*(t405+t6.*(t261-t399));
et17 = dq6.*t1212.*7.263507131821755e+1;
et18 = t6.*(t120-t640+t10.*(dq4.*(t57+t284)+dq3.*t57.*5.110348748545983e-1+t4.*(t328-t331))).*4.126305645247942e-4;
et19 = t11.*(t120-t640+t10.*(dq4.*(t57+t284)+dq3.*t57.*5.110348748545983e-1+t4.*(t328-t331))).*3.146556876441599e-4;
et20 = t6.*(t833-t1063+t1225+dq5.*(t474+t975+t1099)).*7.263507131821755e+1;
et21 = t1188.*(t530-t532+t6.*(t261-t399).*1.336375981993753e+2+t11.*(t261-t399).*7.263507131821755e+1);
t1302 = -t598.*(et16+et17+et18+et19+et20+et21);
et22 = -t567+t609+t6.*(t261-t399).*3.383303336574349e+3;
et23 = t11.*(t261-t399).*1.246862890394724e+3;
et24 = t264+t650.*4.200920957332826e+3+t826+t868+t871-t873+t988+t990-t1089+t1121-t1217+t1247-t1248-t1250-t1251+t1269+t795.*(et22+et23)+t117.*(t405+t6.*(t261-t399));
et25 = dq6.*t1212.*7.263507131821755e+1;
et26 = t6.*(t120-t640+t10.*(dq4.*(t57+t284)+dq3.*t57.*5.110348748545983e-1+t4.*(t328-t331))).*4.126305645247942e-4;
et27 = t11.*(t120-t640+t10.*(dq4.*(t57+t284)+dq3.*t57.*5.110348748545983e-1+t4.*(t328-t331))).*3.146556876441599e-4;
et28 = t6.*(t833-t1063+t1225+dq5.*(t474+t975+t1099)).*7.263507131821755e+1;
et29 = t1188.*(t530-t532+t6.*(t261-t399).*1.336375981993753e+2+t11.*(t261-t399).*7.263507131821755e+1);
t1303 = t598.*(et24+et25+et26+et27+et28+et29);
t1298 = -t1296.*(t311+t6.*(t174-t314));
t1299 = t754.*t1297;
t1300 = t1296.*(t311+t6.*(t174-t314));
et30 = t197-t202+t216-t640.*1.356524863046341e+2+t693-t906-t907+t971-t978+t1107+t1145-t1191-t1192+dq4.*(t57+t284).*4.605359747732407e+2;
et31 = t4.*(t328-t331).*7.092789006718835e+2+t5.*(dq4.*(t57+t284)+dq3.*t57.*5.110348748545983e-1+t4.*(t328-t331)).*6.185536839278779e+1;
et32 = t10.*(dq4.*(t57+t284)+dq3.*t57.*5.110348748545983e-1+t4.*(t328-t331)).*1.356524863046341e+2;
et33 = t78.*(-2.038587093e+1)-t2.*t3.*1.999853938233e+5+t7.*t8.*1.999853938233e+5;
et34 = t12.*(dq1.*3.22231575312482e+2+dq2.*3.22231575312482e+2)+dq1.*t68.*t72;
et35 = t79.*(-2.038587093e+1)+t2.*t8.*1.999853938233e+5+t3.*t7.*1.999853938233e+5;
et36 = -t12.*(dq1.*4.573234736449676e+2+dq2.*4.573234736449676e+2)+dq1.*t68.*t77;
et37 = t85-t763+t935-t9.*t34.*t40.*2.556183965391409e-15;
et38 = -(t211-t222-t744-t781+t899+t968-t1046+t1098.*2.889644336e+1-t1123+t1144+t52.*(t57+t284)+t4.*(t328-t331).*1.328674864713371e+3);
et39 = t2.*(-4.710921170210926e+6)-t7.*2.435931843645872e+7+t73+t74+t75+t76+t169+t170+t1259+t1263+t1265+t1279+t1280+t1285+t1290+t1291+t1293+t1299+t1300+t1303;
et40 = -(t603+t6.*t1163+t11.*(t91-t244-t763+t935)).*(t201+t683+t847+t849+t911+t977+t995+t1022+t1088+t1205+t1216+t1228+t1245+t1267-t66.*(t405+t6.*(t261-t399)))-(t91-t244-t763+t935).*(et30+et31+et32)+t77.*(et33+et34)-t762.*t1242+t934.*t1209-t954.*t1260+t1163.*t1283-t72.*(et35+et36)+et37.*et38+t1286.*(t49+t178+t360+t957+t1082)-t1208.*(t408+t621+t775)+t1282.*(t360+t957+t1082)+t1294.*(t601-t11.*t1163+t6.*(t91-t244-t763+t935));
et41 = t1081.*(t196+t210+t397.*6.678442840618982e+2+t674-t747-t783-t898-t969+t1110-t1124+t1143+t961.*(t96-t333));
et42 = t197-t202+t216-t640.*1.356524863046341e+2+t693-t906-t907+t971-t978+t1107+t1145-t1191-t1192+dq4.*(t57+t284).*4.605359747732407e+2;
et43 = t4.*(t328-t331).*7.092789006718835e+2+t5.*(dq4.*(t57+t284)+dq3.*t57.*5.110348748545983e-1+t4.*(t328-t331)).*6.185536839278779e+1;
et44 = t10.*(dq4.*(t57+t284)+dq3.*t57.*5.110348748545983e-1+t4.*(t328-t331)).*1.356524863046341e+2;
et45 = t85+t773-t9.*t34.*t40.*7.425392937311983e-15;
et46 = -(t211-t222-t744-t781+t899+t968-t1046+t1098.*2.889644336e+1-t1123+t1144+t52.*(t57+t284)+t4.*(t328-t331).*1.328674864713371e+3);
et47 = t73+t74+t75+t76+t169+t170+t1259+t1263+t1265+t1279+t1280+t1285+t1290+t1291+t1293+t1299+t1300+t1303+t1294.*(t601+t6.*t872-t11.*t1064)+t770.*t1209-t775.*t1208-t802.*t1260+t1064.*t1283+t1286.*(t49+t178+t360+t805+t877)+t1282.*(t360+t805+t877)-(t603+t11.*t872+t6.*t1064).*(t201+t683+t847+t849+t911+t977+t995+t1022+t1088+t1205+t1216+t1228+t1245+t1267-t66.*(t405+t6.*(t261-t399)))-t872.*(et42+et43+et44)+et45.*et46;
et48 = t867.*(t196+t210+t397.*6.678442840618982e+2+t674-t747-t783-t898-t969+t1110-t1124+t1143+t961.*(t96-t333))-t34.*t40.*t1242.*4.869208971920574e-15;
et49 = -t567+t609+t6.*(t261-t399).*3.383303336574349e+3;
et50 = t11.*(t261-t399).*1.246862890394724e+3;
et51 = t264+t650.*4.200920957332826e+3+t826+t868+t871-t873+t988+t990-t1089+t1121-t1217+t1247-t1248-t1250-t1251+t1269+t795.*(et49+et50)+t117.*(t405+t6.*(t261-t399));
et52 = dq6.*t1212.*7.263507131821755e+1;
et53 = t6.*(t120-t640+t10.*(dq4.*(t57+t284)+dq3.*t57.*5.110348748545983e-1+t4.*(t328-t331))).*4.126305645247942e-4;
et54 = t11.*(t120-t640+t10.*(dq4.*(t57+t284)+dq3.*t57.*5.110348748545983e-1+t4.*(t328-t331))).*3.146556876441599e-4;
et55 = t6.*(t833-t1063+t1225+dq5.*(t474+t975+t1099)).*7.263507131821755e+1;
et56 = t1188.*(t530-t532+t6.*(t261-t399).*1.336375981993753e+2+t11.*(t261-t399).*7.263507131821755e+1);
et57 = t197-t202+t216-t640.*1.356524863046341e+2+t693-t906-t907+t971-t978+t1107+t1145-t1191-t1192+dq4.*(t57+t284).*4.605359747732407e+2;
et58 = t4.*(t328-t331).*7.092789006718835e+2+t5.*(dq4.*(t57+t284)+dq3.*t57.*5.110348748545983e-1+t4.*(t328-t331)).*6.185536839278779e+1;
et59 = t10.*(dq4.*(t57+t284)+dq3.*t57.*5.110348748545983e-1+t4.*(t328-t331)).*1.356524863046341e+2;
et60 = t266+t267+t280+t293+t558+t563+t640.*7.291450524218959e+2;
et61 = t650.*5.878411097842592e+2+t707+t715+t864+t866+t884+t991+t1002+t1035+t1042+t1076+t1115+t1136+t1158+t1195+t1203+t1237+dq5.*(t474+t975+t1099).*7.051076542399408e-1;
et62 = t397.*3.371409213983255e+2;
et63 = t625.*1.483306048043653e-5;
et64 = t626.*(-8.818711196088817e-6)+t756.*8.595599785252598e-1-t757.*5.110348748545983e-1;
et65 = t800.*(-5.110348748545983e-1)-t801.*8.595599785252598e-1-t806.*8.595599785252598e-1+t809.*5.110348748545983e-1-t908.*5.110348748545983e-1;
et66 = t917.*5.110348748545983e-1-t949.*9.559948463095517e-2;
et67 = t950.*(-8.631091645042425e+1)-t1028.*5.110348748545983e-1+t1029.*8.595599785252598e-1;
et68 = t1051.*8.595599785252598e-1+t1054.*5.110348748545983e-1+t1080.*5.110348748545983e-1;
et69 = t1098.*(-9.559948463095517e-2)+t1101.*8.631091645042425e+1;
et70 = t1128.*(-5.110348748545983e-1)+t1132.*5.110348748545983e-1+t1141.*8.631091645042425e+1;
et71 = t1142.*(-9.559948463095517e-2)+t80.*(et51+et52+et53+et54+et55+et56);
et72 = dq4.*(t57+t284).*(-2.538346896821816)-t887.*(t57+t284).*5.110348748545983e-1;
et73 = -t1286.*(t4.*5.157359871151559+t4.*t5.*4.931128922368695e+1);
et74 = dq3.*t55.*2.159518341551335e+3;
et75 = dq3.*t57.*(-3.498271897117955);
et76 = dq3.*t254.*3.101322990888223e-4;
et77 = dq3.*t257.*(-1.843832014202691e-4);
et78 = dq3.*t765.*(-1.72565741205e-5);
et79 = dq3.*t938.*(-4.586196234965452);
et80 = dq3.*t941.*(-7.713975955870246)-t4.*t1277.*8.595599785252598e-1;
et81 = t9.*t1276.*(-8.595599785252598e-1)-t4.*t1292.*8.595599785252598e-1+t81.*t1287;
et82 = t4.*(t328-t331).*(-4.724604290218056);
et83 = t9.*(t328-t331).*(-2.310978750639558e+3);
et84 = t1294.*(t6.*t9.*4.931128922368695e+1+t6.*t80.*6.0+t4.*t10.*t11.*4.931128922368695e+1)-t1296.*(t4.*t11.*8.595599785252598e-1-t6.*t81);
et85 = -t1297.*(t4.*t6.*8.595599785252598e-1+t11.*t81)-t9.*(et57+et58+et59).*4.931128922368695e+1;
et86 = -(t9.*t11.*4.931128922368695e+1+t11.*t80.*6.0-t4.*t6.*t10.*4.931128922368695e+1).*(t201+t683+t847+t849+t911+t977+t995+t1022+t1088+t1205+t1216+t1228+t1245+t1267-t66.*(t405+t6.*(t261-t399)))+t80.*(et60+et61);
et87 = t4.*(t196+t210+t397.*6.678442840618982e+2+t674-t747-t783-t898-t969+t1110-t1124+t1143+t961.*(t96-t333)).*(-1.291687373922119e+1);
et88 = t9.*(t211-t222-t744-t781+t899+t968-t1046+t1098.*2.889644336e+1-t1123+t1144+t52.*(t57+t284)+t4.*(t328-t331).*1.328674864713371e+3).*(-1.291687373922119e+1);
et89 = dq3.*t12.*t39.*1.680043160985129e+3;
et90 = t34.*t40.*t92.*(-8.564233717611997e-16);
et91 = t34.*t40.*t106.*5.091700655507849e-16;
et92 = t45.*t58.*t92.*1.936876142599284e-6;
et93 = t45.*t58.*t106.*(-3.25782309086522e-6);
et94 = t12.*t39.*t765.*(-4.515804268730207e+1)-t4.*t5.*t1282.*4.931128922368695e+1;
et95 = t4.*t10.*t1283.*(-4.931128922368695e+1);
et96 = -t567+t609+t6.*(t261-t399).*3.383303336574349e+3;
et97 = t11.*(t261-t399).*1.246862890394724e+3;
et98 = t264+t650.*4.200920957332826e+3+t826+t868+t871-t873+t988+t990-t1089+t1121-t1217+t1247-t1248-t1250-t1251+t1269+t795.*(et96+et97)+t117.*(t405+t6.*(t261-t399));
et99 = dq6.*t1212.*7.263507131821755e+1;
et100 = t6.*(t120-t640+t10.*(dq4.*(t57+t284)+dq3.*t57.*5.110348748545983e-1+t4.*(t328-t331))).*4.126305645247942e-4;
et101 = t11.*(t120-t640+t10.*(dq4.*(t57+t284)+dq3.*t57.*5.110348748545983e-1+t4.*(t328-t331))).*3.146556876441599e-4;
et102 = t6.*(t833-t1063+t1225+dq5.*(t474+t975+t1099)).*7.263507131821755e+1;
et103 = t1188.*(t530-t532+t6.*(t261-t399).*1.336375981993753e+2+t11.*(t261-t399).*7.263507131821755e+1);
et104 = t266+t267+t280+t293+t558+t563+t640.*7.291450524218959e+2;
et105 = t650.*5.878411097842592e+2+t707+t715+t864+t866+t884+t991+t1002+t1035+t1042+t1076+t1115+t1136+t1158+t1195+t1203+t1237+dq5.*(t474+t975+t1099).*7.051076542399408e-1;
et106 = t278+t287+t397.*2.92140771649329e+3+t725+t729+t862+t876+t879+t1019-t1024.*6.0-t1026.*6.0+t1049+t1052+t1073+t1162+t1184+t1197+t1198+t1234+t1238.*6.0-dq6.*(t405+t6.*(t261-t399)).*8.018255891962515e+2;
et107 = dq3.*t55.*1.492941226797406e+3+dq6.*t795.*4.358104279093053e+2;
et108 = dq5.*t1164.*(-1.054594745727878e+2)+t5.*t820.*4.465233410425356e+3;
et109 = t6.*t820.*8.018255891962515e+2+t11.*t820.*4.358104279093053e+2+t10.*t1062.*1.054594745727878e+2;
et110 = t5.*t1224.*1.054594745727878e+2+t6.*t1297+t11.*t1296+t6.*(t120-t640+t10.*(dq4.*(t57+t284)+dq3.*t57.*5.110348748545983e-1+t4.*(t328-t331))).*4.358104279093053e+2;
et111 = t11.*(t120-t640+t10.*(dq4.*(t57+t284)+dq3.*t57.*5.110348748545983e-1+t4.*(t328-t331))).*(-8.018255891962515e+2)-t1212.*(t473+t6.*(t261-t399).*7.26735103).*6.0;
et112 = t9.*(t328-t331).*(-2.92140771649329e+3);
et113 = t637.*(t530-t532+t6.*(t261-t399).*1.336375981993753e+2+t11.*(t261-t399).*7.263507131821755e+1).*-6.0;
et114 = -t567+t609+t6.*(t261-t399).*3.383303336574349e+3;
et115 = t11.*(t261-t399).*1.246862890394724e+3;
et116 = t264+t650.*4.200920957332826e+3+t826+t868+t871-t873+t988+t990-t1089+t1121+t1218+t1247-t1248-t1250-t1251+t1269+t795.*(et114+et115)+t117.*(t405+t6.*(t261-t399));
et117 = dq6.*t1211.*(-1.336375981993753e+2);
et118 = t6.*(t120-t640+t10.*(dq4.*(t57+t284)+dq3.*t57.*5.110348748545983e-1+t4.*(t328-t331))).*4.126305645247942e-4;
et119 = t11.*(t120-t640+t10.*(dq4.*(t57+t284)+dq3.*t57.*5.110348748545983e-1+t4.*(t328-t331))).*3.146556876441599e-4;
et120 = t6.*(t833-t1063+t1225+dq5.*(t474+t975+t1099)).*7.263507131821755e+1;
et121 = t1188.*(t530-t532+t6.*(t261-t399).*1.336375981993753e+2+t11.*(t261-t399).*7.263507131821755e+1);
h = real([et39+et40+et41;et47+et48;et62+et63+et64+et65+et66+et67+et68+et69+et70+et71+et72+et73+et74+et75+et76+et77+et78+et79+et80+et81+et82+et83+et84+et85+et86+et87+et88+et89+et90+et91+et92+et93+et94+et95;t1284+t10.*(et98+et99+et100+et101+et102+et103)+t5.*t1287+t10.*(et104+et105)-t10.*t11.*(t201+t683+t847+t849+t911+t977+t995+t1022+t1088+t1205+t1216+t1228+t1245+t1267-t66.*(t405+t6.*(t261-t399))).*6.0+t5.*t6.*t1296+t6.*t10.*t1294.*6.0-t5.*t11.*t1297;et106+et107+et108+et109+et110+et111+et112+et113;et116+et117+et118+et119+et120+et121]);
end
